simulink model "FYI_Twin_CyberResilient"  (R2025b)
settings: Solver=VariableStepAuto  StartTime=0.0  StopTime=TF  FixedStep=1/120  RelTol=1e-5
PreLoadFcn:
  | [aircraft, state] = astDehavillandBeaver();
  | thrustX = getCoefficient(aircraft,"CX","Propeller",Component="Propeller");
model workspace (MATLAB code in the model file + MAT data in the model file):
  ActuatorCmds = [0.0013469; -0.14185; -0.03733]
  AileronCmd = 0.0013469
  ElevatorCmd = -0.14185
  RudderCmd = -0.03733
  TF = 60
  ThrottleCmd = 0.5
  U0 = 33.0529
  V0 = 0.093272
  W0 = 10.1004
  Xe0 = -2.8165e-12
  Ye0 = 4.3033e-12
  Ze0 = -2202
  aircraft = Aero.FixedWing
  aircraft.ReferenceArea = 23.23
  aircraft.ReferenceSpan = 14.63
  aircraft.ReferenceLength = 1.5875
  aircraft.Coefficients = Aero.FixedWing.Coefficient
  aircraft.Coefficients.Values = {-0.0355, 0, 0.0029, 0, 0, 0, 0, 0, 0, 5.459, -5.162, 0, 0, -0.6748, 0, 0; -0.0022, 0, 0, 0, 0, -0.7678, 0, 0, 0, 0, 0, 0, 0, 0, -0.124, 0.3666; -0.055, 0, -5.578, 0, 0, 0, 0, 0, 0, 0, 3.442, 0, 0, -2.988, 0, 0; 0.000591, 0, 0, 0, 0, -0.0618, 0, 0, 0, 0, 0, 0, 0, 0, -0.5045, 0.1695; 0.0945, 0, -0.6028, 0, 0, 0, 0, 0, 0, -2.14, 0, 0.6921, 0, -15.56, 0, -0.3118; -0.0031, 0, 0, 0, 0, 0.0067, 0, 0, 0, 0, 0, 0, 0.1373, 0.1595, -0.1585, -0.1112}
  aircraft.Coefficients.ReferenceFrame = "Body"
  aircraft.Coefficients.StateVariablesInternal = ["Zero" "U" "Alpha" "AlphaDot" "Q" "Beta" "BetaDot" "P" "R" "Alpha2" "Alpha3" "Beta2" "Beta3" "qcV" "pb2V" "rb2V"]
  aircraft.Surfaces(1) = Aero.FixedWing.Surface
  aircraft.Surfaces(1).Surfaces(1) = Aero.FixedWing.Surface
  aircraft.Surfaces(1).Surfaces(1).Coefficients = Aero.FixedWing.Coefficient
  aircraft.Surfaces(1).Surfaces(1).Coefficients.Values = {0, 0; -0.0296, 0; 0, 0; -0.0992, -0.0827; 0, 0; -0.0039, 0}
  aircraft.Surfaces(1).Surfaces(1).Coefficients.ReferenceFrame = "Body"
  aircraft.Surfaces(1).Surfaces(1).Coefficients.StateVariablesInternal = ["Aileron" "AileronAlpha"]
  aircraft.Surfaces(1).Surfaces(1).MaximumValue = 0.523598775598
  aircraft.Surfaces(1).Surfaces(1).MinimumValue = -0.523598775598
  aircraft.Surfaces(1).Surfaces(1).Symmetry = "Symmetric"
  aircraft.Surfaces(1).Surfaces(1).Properties = Aero.Aircraft.Properties
  aircraft.Surfaces(1).Surfaces(1).Properties.Name = "Aileron"
  aircraft.Surfaces(1).Surfaces(2) = Aero.FixedWing.Surface
  aircraft.Surfaces(1).Surfaces(2).Coefficients = Aero.FixedWing.Coefficient
  aircraft.Surfaces(1).Surfaces(2).Coefficients.Values = {-0.0945, 1.106; 0, 0; -1.377, -1.261; 0, 0; 0.4072, 0; 0, 0}
  aircraft.Surfaces(1).Surfaces(2).Coefficients.ReferenceFrame = "Body"
  aircraft.Surfaces(1).Surfaces(2).Coefficients.StateVariablesInternal = ["Flap" "FlapAlpha"]
  aircraft.Surfaces(1).Surfaces(2).MaximumValue = 0.523598775598
  aircraft.Surfaces(1).Surfaces(2).MinimumValue = -0.523598775598
  aircraft.Surfaces(1).Surfaces(2).Symmetry = "Symmetric"
  aircraft.Surfaces(1).Surfaces(2).Properties = Aero.Aircraft.Properties
  aircraft.Surfaces(1).Surfaces(2).Properties.Name = "Flap"
  aircraft.Surfaces(1).Controllable : enumeration (value not decoded)
  aircraft.Surfaces(1).Symmetry = "Symmetric"
  aircraft.Surfaces(1).Properties = Aero.Aircraft.Properties
  aircraft.Surfaces(1).Properties.Name = "Wing"
  aircraft.Surfaces(2) = Aero.FixedWing.Surface
  aircraft.Surfaces(2).Surfaces = Aero.FixedWing.Surface
  aircraft.Surfaces(2).Surfaces.Coefficients = Aero.FixedWing.Coefficient
  aircraft.Surfaces(2).Surfaces.Coefficients.Values = {0, 0; 0, 0; -0.398, -15.93; 0, 0; -1.921, 0; 0, 0}
  aircraft.Surfaces(2).Surfaces.Coefficients.ReferenceFrame = "Body"
  aircraft.Surfaces(2).Surfaces.Coefficients.StateVariablesInternal = ["Elevator" "ElevatorBeta2"]
  aircraft.Surfaces(2).Surfaces.MaximumValue = 0.523598775598
  aircraft.Surfaces(2).Surfaces.MinimumValue = -0.523598775598
  aircraft.Surfaces(2).Surfaces.Symmetry = "Symmetric"
  aircraft.Surfaces(2).Surfaces.Properties = Aero.Aircraft.Properties
  aircraft.Surfaces(2).Surfaces.Properties.Name = "Elevator"
  aircraft.Surfaces(2).Controllable : enumeration (value not decoded)
  aircraft.Surfaces(2).Symmetry = "Symmetric"
  aircraft.Surfaces(2).Properties = Aero.Aircraft.Properties
  aircraft.Surfaces(2).Properties.Name = "HorizontalStabilizer"
  aircraft.Surfaces(3) = Aero.FixedWing.Surface
  aircraft.Surfaces(3).Surfaces = Aero.FixedWing.Surface
  aircraft.Surfaces(3).Surfaces.Coefficients = Aero.FixedWing.Coefficient
  aircraft.Surfaces(3).Surfaces.Coefficients.Values = {0.0341, 0; 0.1158, 0.5238; 0, 0; 0.0069, 0; 0, 0; -0.0827, 0}
  aircraft.Surfaces(3).Surfaces.Coefficients.ReferenceFrame = "Body"
  aircraft.Surfaces(3).Surfaces.Coefficients.StateVariablesInternal = ["Rudder" "RudderAlpha"]
  aircraft.Surfaces(3).Surfaces.MaximumValue = 1.0471975512
  aircraft.Surfaces(3).Surfaces.MinimumValue = -1.0471975512
  aircraft.Surfaces(3).Surfaces.Symmetry = "Symmetric"
  aircraft.Surfaces(3).Surfaces.Properties = Aero.Aircraft.Properties
  aircraft.Surfaces(3).Surfaces.Properties.Name = "Rudder"
  aircraft.Surfaces(3).Controllable : enumeration (value not decoded)
  aircraft.Surfaces(3).Symmetry = "Symmetric"
  aircraft.Surfaces(3).Properties = Aero.Aircraft.Properties
  aircraft.Surfaces(3).Properties.Name = "VerticalStabilizer"
  aircraft.Thrusts = Aero.FixedWing.Thrust
  aircraft.Thrusts.Coefficients = Aero.FixedWing.Coefficient
  aircraft.Thrusts.Coefficients.Values{1} = Simulink.LookupTable
  aircraft.Thrusts.Coefficients.Values{1}.Table = Simulink.lookuptable.Table
  aircraft.Thrusts.Coefficients.Values{1}.Table.Value = [11.3740665205 82.7365658256 548.333441302 2300 4051.6665587 4517.26343417 4588.62593348]
  aircraft.Thrusts.Coefficients.Values{1}.Table.Dimensions = [1 7]
  aircraft.Thrusts.Coefficients.Values{1}.Table.DataType = 'auto'
  aircraft.Thrusts.Coefficients.Values{1}.Table.FieldName = 'Table'
  aircraft.Thrusts.Coefficients.Values{1}.Breakpoints = Simulink.lookuptable.Breakpoint
  aircraft.Thrusts.Coefficients.Values{1}.Breakpoints.Value = [0 0.166666666667 0.333333333333 0.5 0.666666666667 0.833333333333 1]
  aircraft.Thrusts.Coefficients.Values{1}.Breakpoints.TunableSizeName = 'N1'
  aircraft.Thrusts.Coefficients.Values{1}.Breakpoints.TunableSizeValue = -1
  aircraft.Thrusts.Coefficients.Values{1}.Breakpoints.Dimensions = [1 7]
  aircraft.Thrusts.Coefficients.Values{1}.Breakpoints.DataType = 'auto'
  aircraft.Thrusts.Coefficients.Values{1}.Breakpoints.FieldName = 'Propeller'
  aircraft.Thrusts.Coefficients.Values{1}.AllowMultipleInstancesOfTypeToHaveDifferentTableBreakpointSizes = 0
  aircraft.Thrusts.Coefficients.Values{1}.SupportTunableSize = 0
  aircraft.Thrusts.Coefficients.Values{1}.StructTypeInfo = Simulink.lookuptable.StructTypeInfo
  aircraft.Thrusts.Coefficients.Values{1}.StructTypeInfo.Name = 'Dehavilland_Beaver_Propeller_CX_Propeller'
  aircraft.Thrusts.Coefficients.Values{1}.StructTypeInfo.DataScope = 'Auto'
  aircraft.Thrusts.Coefficients.Values{2} = 0
  aircraft.Thrusts.Coefficients.Values{3} = 0
  aircraft.Thrusts.Coefficients.Values{4} = 0
  aircraft.Thrusts.Coefficients.Values{5} = 0
  aircraft.Thrusts.Coefficients.Values{6} = 0
  aircraft.Thrusts.Coefficients.ReferenceFrame = "Body"
  aircraft.Thrusts.Coefficients.MultiplyStateVariables : enumeration (value not decoded)
  aircraft.Thrusts.Coefficients.NonDimensional : enumeration (value not decoded)
  aircraft.Thrusts.Coefficients.StateVariablesInternal = "Propeller"
  aircraft.Thrusts.MaximumValue = 1
  aircraft.Thrusts.MinimumValue = 0
  aircraft.Thrusts.Symmetry = "Symmetric"
  aircraft.Thrusts.Properties = Aero.Aircraft.Properties
  aircraft.Thrusts.Properties.Name = "Propeller"
  aircraft.Properties = Aero.Aircraft.Properties
  aircraft.Properties.Name = "Dehavilland_Beaver"
  aircraft.Properties.Description = "Dehavilland Beaver demo"
  aircraft.Properties.Type = "General Aviation"
  aircraft.Properties.Version = "1.0"
  aircraft.TemperatureSystem = "Kelvin"
  altitude0 = 2202
  attack_enable = 1
  attack_mode = 3
  blend_rate = 0.05
  inputs0.time = 0
  inputs0.signals(1).dimensions = 1
  inputs0.signals(1).values = -0.104711430294
  inputs0.signals(2).dimensions = 1
  inputs0.signals(2).values = -0.0698725229544
  inputs0.signals(3).dimensions = 1
  inputs0.signals(3).values = -0.000215042330254
  lat0 = 0.843936506509
  lat0_deg = 48.354
  lon0 = 0.205746393542
  lon0_deg = 11.7884
  p0 = 3.0707e-20
  phi0 = 0.0092342
  psi0 = 0
  q0 = 5.1124e-22
  r0 = -8.6217e-20
  required_count = 5
  state = astDehavillandBeaverState
  state.Mass = 2288.231
  state.Inertia = table
  state.Inertia.data = {[5788; 0; -117.6], [0; 6928.9; 0], [117.6; 0; 11578.3]}
  state.Inertia.ndims = 2
  state.Inertia.nrows = 3
  state.Inertia.rownames = {'X'; 'Y'; 'Z'}
  state.Inertia.nvars = 3
  state.Inertia.varnames = {'X', 'Y', 'Z'}
  state.Inertia.props.CustomProps = struct()
  state.Inertia.props.VariableCustomProps = struct()
  state.Inertia.props.versionSavedFrom = 5
  state.Inertia.props.minCompatibleVersion = 1
  state.Inertia.props.incompatibilityMsg = ''
  state.Inertia.props.VersionSavedFrom = 5
  state.Inertia.props.useVariableNamesOriginal = 0
  state.Inertia.props.useVariableNames2048 = 0
  state.Inertia.props.useDimensionNamesOriginal = 0
  state.Inertia.props.useDimensionNames2048 = 0
  state.Inertia.props.Description = ''
  state.Inertia.props.VariableNamesOriginal = {}
  state.Inertia.props.VariableNames2048 = {}
  state.Inertia.props.DimensionNames = {'Row', 'Variables'}
  state.Inertia.props.DimensionNamesOriginal = {}
  state.Inertia.props.DimensionNames2048 = {}
  state.Inertia.props.UserData = []
  state.Inertia.props.VariableDescriptions = {}
  state.Inertia.props.VariableUnits = {}
  state.Inertia.props.VariableContinuity = {}
  state.AltitudeMSL = 2202
  state.XN = -2.8165e-12
  state.XE = 4.3033e-12
  state.U = 33.0529
  state.V = 0.093272
  state.W = 10.1004
  state.Phi = 0.0092342
  state.Theta = 0.29658
  state.P = 3.0707e-20
  state.Q = 5.1124e-22
  state.R = -8.6217e-20
  state.Environment = Aero.Aircraft.Environment
  state.Environment.Density = 0.986207191626
  state.Environment.Temperature = 273.837
  state.Environment.Pressure = 77521.5580145
  state.Environment.SpeedOfSound = 331.734913638
  state.ControlStates(1) = Aero.Aircraft.ControlState
  state.ControlStates(1).MaximumValue = 0.523598775598
  state.ControlStates(1).MinimumValue = -0.523598775598
  state.ControlStates(1).PositionInternal = 0.0091
  state.ControlStates(1).Properties = Aero.Aircraft.Properties
  state.ControlStates(1).Properties.Name = "Aileron"
  state.ControlStates(2) = Aero.Aircraft.ControlState
  state.ControlStates(2).MaximumValue = 0.523598775598
  state.ControlStates(2).MinimumValue = -0.523598775598
  state.ControlStates(2).Properties = Aero.Aircraft.Properties
  state.ControlStates(2).Properties.Name = "Flap"
  state.ControlStates(3) = Aero.Aircraft.ControlState
  state.ControlStates(3).MaximumValue = 0.523598775598
  state.ControlStates(3).MinimumValue = -0.523598775598
  state.ControlStates(3).PositionInternal = -0.0425
  state.ControlStates(3).Properties = Aero.Aircraft.Properties
  state.ControlStates(3).Properties.Name = "Elevator"
  state.ControlStates(4) = Aero.Aircraft.ControlState
  state.ControlStates(4).MaximumValue = 1.0471975512
  state.ControlStates(4).MinimumValue = -1.0471975512
  state.ControlStates(4).PositionInternal = -0.046
  state.ControlStates(4).Properties = Aero.Aircraft.Properties
  state.ControlStates(4).Properties.Name = "Rudder"
  state.ControlStates(5) = Aero.Aircraft.ControlState
  state.ControlStates(5).MaximumValue = 1
  state.ControlStates(5).MinimumValue = 0
  state.ControlStates(5).DeflectionAngle : enumeration (value not decoded)
  state.ControlStates(5).PositionInternal = 0.5
  state.ControlStates(5).Properties = Aero.Aircraft.Properties
  state.ControlStates(5).Properties.Name = "Propeller"
  state.TemperatureSystem = "Kelvin"
  states.time = 0
  states.signals(1).values = 0
  states.signals(1).dimensions = 1
  states.signals(1).label = 'CSTATE'
  states.signals(1).blockName = 'asb6DOFAirframeTemplate/6DOF EOM/6DOF (Euler Angles)/xe,ye,ze'
  states.signals(1).stateName = 'Xe'
  states.signals(1).inReferencedModel = 0
  states.signals(1).sampleTime = [0 0]
  states.signals(2).values = 0
  states.signals(2).dimensions = 1
  states.signals(2).label = 'CSTATE'
  states.signals(2).blockName = 'asb6DOFAirframeTemplate/6DOF EOM/6DOF (Euler Angles)/xe,ye,ze'
  states.signals(2).stateName = 'Ye'
  states.signals(2).inReferencedModel = 0
  states.signals(2).sampleTime = [0 0]
  states.signals(3).values = -2202
  states.signals(3).dimensions = 1
  states.signals(3).label = 'CSTATE'
  states.signals(3).blockName = 'asb6DOFAirframeTemplate/6DOF EOM/6DOF (Euler Angles)/xe,ye,ze'
  states.signals(3).stateName = 'Ze'
  states.signals(3).inReferencedModel = 0
  states.signals(3).sampleTime = [0 0]
  states.signals(4).values = 0.128665353089
  states.signals(4).dimensions = 1
  states.signals(4).label = 'CSTATE'
  states.signals(4).blockName = 'asb6DOFAirframeTemplate/6DOF EOM/6DOF (Euler Angles)/Calculate DCM &
    | Euler Angles/phi
    | theta
    | psi'
  states.signals(4).stateName = 'phi'
  states.signals(4).inReferencedModel = 0
  states.signals(4).sampleTime = [0 0]
  states.signals(5).values = 0.259337659946
  states.signals(5).dimensions = 1
  states.signals(5).label = 'CSTATE'
  states.signals(5).blockName = 'asb6DOFAirframeTemplate/6DOF EOM/6DOF (Euler Angles)/Calculate DCM &
    | Euler Angles/phi
    | theta
    | psi'
  states.signals(5).stateName = 'theta'
  states.signals(5).inReferencedModel = 0
  states.signals(5).sampleTime = [0 0]
  states.signals(6).values = -0.178947917154
  states.signals(6).dimensions = 1
  states.signals(6).label = 'CSTATE'
  states.signals(6).blockName = 'asb6DOFAirframeTemplate/6DOF EOM/6DOF (Euler Angles)/Calculate DCM &
    | Euler Angles/phi
    | theta
    | psi'
  states.signals(6).stateName = 'psi'
  states.signals(6).inReferencedModel = 0
  states.signals(6).sampleTime = [0 0]
  states.signals(7).values = 36.9119692666
  states.signals(7).dimensions = 1
  states.signals(7).label = 'CSTATE'
  states.signals(7).blockName = 'asb6DOFAirframeTemplate/6DOF EOM/6DOF (Euler Angles)/ub,vb,wb'
  states.signals(7).stateName = 'Ubody'
  states.signals(7).inReferencedModel = 0
  states.signals(7).sampleTime = [0 0]
  states.signals(8).values = 8.10720863264
  states.signals(8).dimensions = 1
  states.signals(8).label = 'CSTATE'
  states.signals(8).blockName = 'asb6DOFAirframeTemplate/6DOF EOM/6DOF (Euler Angles)/ub,vb,wb'
  states.signals(8).stateName = 'Vbody'
  states.signals(8).inReferencedModel = 0
  states.signals(8).sampleTime = [0 0]
  states.signals(9).values = 8.82591882596
  states.signals(9).dimensions = 1
  states.signals(9).label = 'CSTATE'
  states.signals(9).blockName = 'asb6DOFAirframeTemplate/6DOF EOM/6DOF (Euler Angles)/ub,vb,wb'
  states.signals(9).stateName = 'Wbody'
  states.signals(9).inReferencedModel = 0
  states.signals(9).sampleTime = [0 0]
  states.signals(10).values = 0
  states.signals(10).dimensions = 1
  states.signals(10).label = 'CSTATE'
  states.signals(10).blockName = 'asb6DOFAirframeTemplate/6DOF EOM/6DOF (Euler Angles)/p,q,r '
  states.signals(10).stateName = 'p'
  states.signals(10).inReferencedModel = 0
  states.signals(10).sampleTime = [0 0]
  states.signals(11).values = 0
  states.signals(11).dimensions = 1
  states.signals(11).label = 'CSTATE'
  states.signals(11).blockName = 'asb6DOFAirframeTemplate/6DOF EOM/6DOF (Euler Angles)/p,q,r '
  states.signals(11).stateName = 'q'
  states.signals(11).inReferencedModel = 0
  states.signals(11).sampleTime = [0 0]
  states.signals(12).values = 0
  states.signals(12).dimensions = 1
  states.signals(12).label = 'CSTATE'
  states.signals(12).blockName = 'asb6DOFAirframeTemplate/6DOF EOM/6DOF (Euler Angles)/p,q,r '
  states.signals(12).stateName = 'r'
  states.signals(12).inReferencedModel = 0
  states.signals(12).sampleTime = [0 0]
  states.signals(13).values = [0 0]
  states.signals(13).dimensions = 2
  states.signals(13).label = 'CSTATE'
  states.signals(13).blockName = 'asb6DOFAirframeTemplate/Environment Model/Dryden Wind Turbulence Model 
    | (Continuous (+q +r))/Filters on velocities/Hwgw(s)/wg_p1'
  states.signals(13).stateName = ''
  states.signals(13).inReferencedModel = 0
  states.signals(13).sampleTime = [0 0]
  states.signals(14).values = [0 0]
  states.signals(14).dimensions = 2
  states.signals(14).label = 'CSTATE'
  states.signals(14).blockName = 'asb6DOFAirframeTemplate/Environment Model/Dryden Wind Turbulence Model 
    | (Continuous (+q +r))/Filters on velocities/Hwgw(s)/wg_p2'
  states.signals(14).stateName = ''
  states.signals(14).inReferencedModel = 0
  states.signals(14).sampleTime = [0 0]
  states.signals(15).values = [0 0]
  states.signals(15).dimensions = 2
  states.signals(15).label = 'CSTATE'
  states.signals(15).blockName = 'asb6DOFAirframeTemplate/Environment Model/Dryden Wind Turbulence Model 
    | (Continuous (+q +r))/Filters on velocities/Hvgw(s)/vg_p1'
  states.signals(15).stateName = ''
  states.signals(15).inReferencedModel = 0
  states.signals(15).sampleTime = [0 0]
  states.signals(16).values = [0 0]
  states.signals(16).dimensions = 2
  states.signals(16).label = 'CSTATE'
  states.signals(16).blockName = 'asb6DOFAirframeTemplate/Environment Model/Dryden Wind Turbulence Model 
    | (Continuous (+q +r))/Filters on velocities/Hvgw(s)/vgw_p2'
  states.signals(16).stateName = ''
  states.signals(16).inReferencedModel = 0
  states.signals(16).sampleTime = [0 0]
  states.signals(17).values = [0 0]
  states.signals(17).dimensions = 2
  states.signals(17).label = 'CSTATE'
  states.signals(17).blockName = 'asb6DOFAirframeTemplate/Environment Model/Dryden Wind Turbulence Model 
    | (Continuous (+q +r))/Filters on velocities/Hugw(s)/ug_p'
  states.signals(17).stateName = ''
  states.signals(17).inReferencedModel = 0
  states.signals(17).sampleTime = [0 0]
  states.signals(18).values = [0 0]
  states.signals(18).dimensions = 2
  states.signals(18).label = 'CSTATE'
  states.signals(18).blockName = 'asb6DOFAirframeTemplate/Environment Model/Dryden Wind Turbulence Model 
    | (Continuous (+q +r))/Filters on angular rates/Hrgw/rgw_p'
  states.signals(18).stateName = ''
  states.signals(18).inReferencedModel = 0
  states.signals(18).sampleTime = [0 0]
  states.signals(19).values = [0 0]
  states.signals(19).dimensions = 2
  states.signals(19).label = 'CSTATE'
  states.signals(19).blockName = 'asb6DOFAirframeTemplate/Environment Model/Dryden Wind Turbulence Model 
    | (Continuous (+q +r))/Filters on angular rates/Hqgw/qgw_p'
  states.signals(19).stateName = ''
  states.signals(19).inReferencedModel = 0
  states.signals(19).sampleTime = [0 0]
  states.signals(20).values = [0 0]
  states.signals(20).dimensions = 2
  states.signals(20).label = 'CSTATE'
  states.signals(20).blockName = 'asb6DOFAirframeTemplate/Environment Model/Dryden Wind Turbulence Model 
    | (Continuous (+q +r))/Filters on angular rates/Hpgw/pgw_p'
  states.signals(20).stateName = ''
  states.signals(20).inReferencedModel = 0
  states.signals(20).sampleTime = [0 0]
  states0.time = 0
  states0.signals(1).values = [0 0 -2202]
  states0.signals(1).dimensions = 3
  states0.signals(1).label = 'CSTATE'
  states0.signals(1).blockName = 'asb6DOFAirframeTemplate/6DOF EOM/6DOF (Euler Angles)/xe,ye,ze'
  states0.signals(1).stateName = ''
  states0.signals(1).inReferencedModel = 0
  states0.signals(1).sampleTime = [0 0]
  states0.signals(2).values = [0.128665353089 0.259337659946 -0.178947917154]
  states0.signals(2).dimensions = 3
  states0.signals(2).label = 'CSTATE'
  states0.signals(2).blockName = 'asb6DOFAirframeTemplate/6DOF EOM/6DOF (Euler Angles)/Calculate DCM &
    | Euler Angles/phi
    | theta
    | psi'
  states0.signals(2).stateName = ''
  states0.signals(2).inReferencedModel = 0
  states0.signals(2).sampleTime = [0 0]
  states0.signals(3).values = [36.9119692666 8.10720863264 8.82591882596]
  states0.signals(3).dimensions = 3
  states0.signals(3).label = 'CSTATE'
  states0.signals(3).blockName = 'asb6DOFAirframeTemplate/6DOF EOM/6DOF (Euler Angles)/ub,vb,wb'
  states0.signals(3).stateName = ''
  states0.signals(3).inReferencedModel = 0
  states0.signals(3).sampleTime = [0 0]
  states0.signals(4).values = [0 0 0]
  states0.signals(4).dimensions = 3
  states0.signals(4).label = 'CSTATE'
  states0.signals(4).blockName = 'asb6DOFAirframeTemplate/6DOF EOM/6DOF (Euler Angles)/p,q,r '
  states0.signals(4).stateName = ''
  states0.signals(4).inReferencedModel = 0
  states0.signals(4).sampleTime = [0 0]
  states0.signals(5).values = [0 0]
  states0.signals(5).dimensions = 2
  states0.signals(5).label = 'CSTATE'
  states0.signals(5).blockName = 'asb6DOFAirframeTemplate/Environment Model/Dryden Wind Turbulence Model 
    | (Continuous (+q +r))/Filters on velocities/Hwgw(s)/wg_p1'
  states0.signals(5).stateName = ''
  states0.signals(5).inReferencedModel = 0
  states0.signals(5).sampleTime = [0 0]
  states0.signals(6).values = [0 0]
  states0.signals(6).dimensions = 2
  states0.signals(6).label = 'CSTATE'
  states0.signals(6).blockName = 'asb6DOFAirframeTemplate/Environment Model/Dryden Wind Turbulence Model 
    | (Continuous (+q +r))/Filters on velocities/Hwgw(s)/wg_p2'
  states0.signals(6).stateName = ''
  states0.signals(6).inReferencedModel = 0
  states0.signals(6).sampleTime = [0 0]
  states0.signals(7).values = [0 0]
  states0.signals(7).dimensions = 2
  states0.signals(7).label = 'CSTATE'
  states0.signals(7).blockName = 'asb6DOFAirframeTemplate/Environment Model/Dryden Wind Turbulence Model 
    | (Continuous (+q +r))/Filters on velocities/Hvgw(s)/vg_p1'
  states0.signals(7).stateName = ''
  states0.signals(7).inReferencedModel = 0
  states0.signals(7).sampleTime = [0 0]
  states0.signals(8).values = [0 0]
  states0.signals(8).dimensions = 2
  states0.signals(8).label = 'CSTATE'
  states0.signals(8).blockName = 'asb6DOFAirframeTemplate/Environment Model/Dryden Wind Turbulence Model 
    | (Continuous (+q +r))/Filters on velocities/Hvgw(s)/vgw_p2'
  states0.signals(8).stateName = ''
  states0.signals(8).inReferencedModel = 0
  states0.signals(8).sampleTime = [0 0]
  states0.signals(9).values = [0 0]
  states0.signals(9).dimensions = 2
  states0.signals(9).label = 'CSTATE'
  states0.signals(9).blockName = 'asb6DOFAirframeTemplate/Environment Model/Dryden Wind Turbulence Model 
    | (Continuous (+q +r))/Filters on velocities/Hugw(s)/ug_p'
  states0.signals(9).stateName = ''
  states0.signals(9).inReferencedModel = 0
  states0.signals(9).sampleTime = [0 0]
  states0.signals(10).values = [0 0]
  states0.signals(10).dimensions = 2
  states0.signals(10).label = 'CSTATE'
  states0.signals(10).blockName = 'asb6DOFAirframeTemplate/Environment Model/Dryden Wind Turbulence Model 
    | (Continuous (+q +r))/Filters on angular rates/Hrgw/rgw_p'
  states0.signals(10).stateName = ''
  states0.signals(10).inReferencedModel = 0
  states0.signals(10).sampleTime = [0 0]
  states0.signals(11).values = [0 0]
  states0.signals(11).dimensions = 2
  states0.signals(11).label = 'CSTATE'
  states0.signals(11).blockName = 'asb6DOFAirframeTemplate/Environment Model/Dryden Wind Turbulence Model 
    | (Continuous (+q +r))/Filters on angular rates/Hqgw/qgw_p'
  states0.signals(11).stateName = ''
  states0.signals(11).inReferencedModel = 0
  states0.signals(11).sampleTime = [0 0]
  states0.signals(12).values = [0 0]
  states0.signals(12).dimensions = 2
  states0.signals(12).label = 'CSTATE'
  states0.signals(12).blockName = 'asb6DOFAirframeTemplate/Environment Model/Dryden Wind Turbulence Model 
    | (Continuous (+q +r))/Filters on angular rates/Hpgw/pgw_p'
  states0.signals(12).stateName = ''
  states0.signals(12).inReferencedModel = 0
  states0.signals(12).sampleTime = [0 0]
  theta0 = 0.29658
  thrustX = Simulink.LookupTable
  thrustX.Table = Simulink.lookuptable.Table
  thrustX.Table.Value = [11.3740665205 82.7365658256 548.333441302 2300 4051.6665587 4517.26343417 4588.62593348]
  thrustX.Table.Dimensions = [1 7]
  thrustX.Table.DataType = 'auto'
  thrustX.Table.FieldName = 'Table'
  thrustX.Breakpoints = Simulink.lookuptable.Breakpoint
  thrustX.Breakpoints.Value = [0 0.166666666667 0.333333333333 0.5 0.666666666667 0.833333333333 1]
  thrustX.Breakpoints.TunableSizeName = 'N1'
  thrustX.Breakpoints.TunableSizeValue = -1
  thrustX.Breakpoints.Dimensions = [1 7]
  thrustX.Breakpoints.DataType = 'auto'
  thrustX.Breakpoints.FieldName = 'Propeller'
  thrustX.AllowMultipleInstancesOfTypeToHaveDifferentTableBreakpointSizes = 0
  thrustX.SupportTunableSize = 0
  thrustX.StructTypeInfo = Simulink.lookuptable.StructTypeInfo
  thrustX.StructTypeInfo.Name = 'Dehavilland_Beaver_Propeller_CX_Propeller'
  thrustX.StructTypeInfo.DataScope = 'Auto'
  u_twin = [0.0013469; -0.14185; -0.03733; 0.5; 0.5]
  x0 = [0.0092342; 0.29658; 0; 3.0707e-20; 5.1124e-22; -8.6217e-20; 33.0529; 0.093272; 10.1004; -2.8165e-12; 4.3033e-12; -2202]
  x0_beaver = [0.0092342; 0.29658; 0; 3.0707e-20; 5.1124e-22; -8.6217e-20; 33.0529; 0.093272; 10.1004; -2.8165e-12; 4.3033e-12; -8202]
  x0_unified = [33.0529; 0.093272; 10.1004; 0.0092342; 0.29658; 0; 3.0707e-20; 5.1124e-22; -8.6217e-20; 0.205746393542; 0.843936506509; 2202]
  other statements: initialize6DOFSkyHogg;
undefined symbols (not defined in the file or in its folder): F, Light, MIL
libraries: aerolibasang x6, aerolibobsolete x2, aerolibadyn x2, aerolibatmos2 x2, aerolibwind2 x2, sharedtransform x2, aerolibfltsims x2
(part 1 of 2)
settings Model: Creator=admin2025  LastModifiedBy=admin2025
settings SolverCC: AlgebraicLoopSolver=TrustRegion  AutoInsertRateTranBlk=on  InsertRTBMode=Never (minimum delay)  MinimalZcImpactIntegration=on  MaxZcPerStep=1.0
settings DataIOCC: ExternalInput=inputs0  InitialState=states  SaveFormat=Array  SaveOutput=off
settings OptimizationCC: BlockReduction=off  EnhancedBackFolding=on  StrengthReduction=on  InitFltsAndDblsToZero=on  DifferentSizesBufferReuse=on
settings DebuggingCC: WriteAfterWriteMsg=DisableAll  AlgebraicLoopMsg=none  FcnCallInpInsideContextMsg=warning  UniqueDataStoreMsg=error  RootOutportRequireBusObject=none  StateNameClashWarn=warning  StrictBusMsg=ErrorOnBusTreatedAsVector  SFUnexpectedBacktrackingDiag=warning  SFNoUnconditionalDefaultTransitionDiag=warning  SFExecutionAtInitializationDiag=none  ArithmeticOperatorsInVariantConditions=warning
settings ModelReferenceCC: EnableRefExpFcnMdlSchedulingChecks=on  PropagateSignalLabelsOutOfModel=off
settings SFSimCC: SimUseLocalCustomCode=off
settings RTWCC: RTWUseLocalCustomCode=off  GPUComputeCapability=3.5  DLArmComputeVersion=19.05
settings CodeAppCC: StateflowObjectComments=on

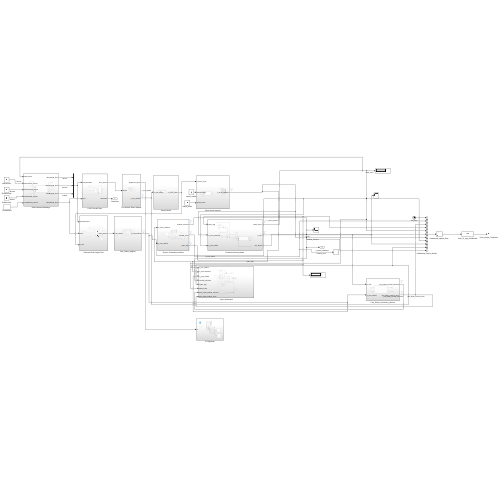
[thumbnail: Simulink's stored preview of the top-level diagram]
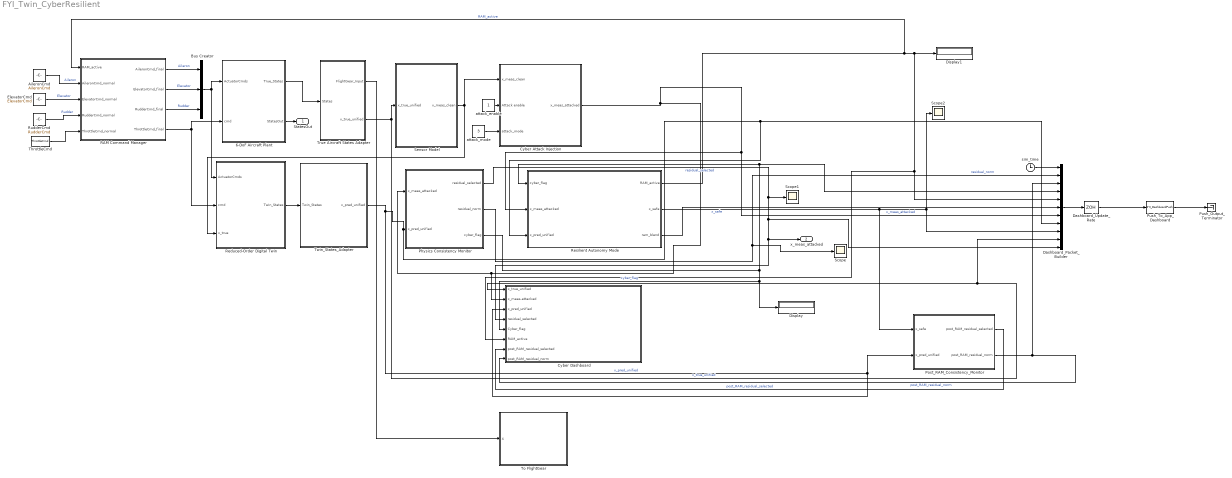
== system FYI_Twin_CyberResilient ==
  6-DoF Aircraft Plant : Subsystem
  AileronCmd : Constant  Value=AileronCmd
  Bus Creator : BusCreator  Inputs=3
  Cyber Attack Injection : Subsystem
  Cyber Dashboard : Subsystem
  Dashboard_Packet_Builder : Concatenate  NumInputs=11
  Dashboard_Update_Rate : ZeroOrderHold  SampleTime=0.1
  Display : Display
  Display1 : Display
  ElevatorCmd : Constant  Value=ElevatorCmd
  Physics Consistency Monitor : Subsystem
  Post_RAM_Consistency_Monitor : Subsystem
  Push_Output_Terminator : Terminator
  Push_To_App_Dashboard : MATLABFcn  MATLABFcn=FYI_DashboardPush
  RAM Command Manager : Subsystem
  Reduced-Order Digital Twin : Subsystem
  Resilient Autonomy Mode : Subsystem
  RudderCmd : Constant  Value=RudderCmd
  Scope : Scope
      settings: ActiveDisplayYMinimum=-76.842271512465658  ActiveDisplayYMaximum=252.07105432729637
  Scope1 : Scope
      settings: ActiveDisplayYMinimum=-7003.9392800862915  ActiveDisplayYMaximum=32762.478212818387  DataLoggingVariableName=ScopeData2
  Scope2 : Scope
      settings: ActiveDisplayYMinimum=-156.7497759524484  ActiveDisplayYMaximum=421.4820575637267  DataLoggingVariableName=ScopeData3
  Sensor Model : Subsystem
  ThrottleCmd : Constant  Value=ThrottleCmd
  To FlightGear : Subsystem
  True Aircraft States Adapter : Subsystem
  Twin_States_Adapter : Subsystem
  attack_enable : Constant
  attack_mode : Constant  Value=3
  sim_time : Clock
  StatesOut : Outport  OutDataTypeStr=double  VectorParamsAs1DForOutWhenUnconnected=off
  x_meas_attacked : Outport  Port=2
  wires:
  6-DoF Aircraft Plant/1(True_States) -> True Aircraft States Adapter/1(States)
  Bus Creator/1 -> 6-DoF Aircraft Plant/1(ActuatorCmds), Reduced-Order Digital Twin/1(ActuatorCmds)
  6-DoF Aircraft Plant/2(StatesOut) -> StatesOut/1
  Sensor Model/1(x_meas_clean) -> Reduced-Order Digital Twin/3(x_true), Cyber Attack Injection/1(x_meas_clean)
  Cyber Attack Injection/1(x_meas_attacked) -> Dashboard_Packet_Builder/7, Resilient Autonomy Mode/2(x_meas_attacked), Physics Consistency Monitor/1(x_meas_attacked), Cyber Dashboard/2(x_meas-attacked)  "x_meas_attacked"
  Physics Consistency Monitor/1(residual_selected) -> Cyber Dashboard/4(residual_selected), x_meas_attacked/1, Dashboard_Packet_Builder/11, Scope1/1  "residual_selected"
  Twin_States_Adapter/1(x_pred_unified) -> Cyber Dashboard/3(x_pred_unified), Post_RAM_Consistency_Monitor/2(x_pred_unified), Dashboard_Packet_Builder/8, Resilient Autonomy Mode/3(x_pred_unified), Physics Consistency Monitor/2(x_pred_unified)  "x_pred_unified"
  True Aircraft States Adapter/2(x_true_unified) -> Sensor Model/1(x_true_unified), Dashboard_Packet_Builder/10, Cyber Dashboard/1(x_true_unified)  "x_true_unified"
  attack_enable/1 -> Cyber Attack Injection/2(Attack enable)
  Physics Consistency Monitor/2(residual_norm) -> Dashboard_Packet_Builder/2, Scope/1  "residual_norm"
  Physics Consistency Monitor/3(cyber_flag) -> Dashboard_Packet_Builder/4, Resilient Autonomy Mode/1(cyber_flag), Display/1, Cyber Dashboard/5(Cyber_flag)  "cyber_flag"
  Resilient Autonomy Mode/2(x_safe) -> Scope2/1, Dashboard_Packet_Builder/9, Post_RAM_Consistency_Monitor/1(x_safe)  "x_safe"
  Resilient Autonomy Mode/1(RAM_active) -> Cyber Dashboard/6(RAM_active), Dashboard_Packet_Builder/5, Display1/1, RAM Command Manager/1(RAM_active)  "RAM_active"
  attack_mode/1 -> Cyber Attack Injection/3(attack_mode)
  AileronCmd/1 -> RAM Command Manager/2(AileronCmd_normal)  "Aileron"
  RAM Command Manager/1(AileronCmd_final) -> Bus Creator/1  "Aileron"
  ElevatorCmd/1 -> RAM Command Manager/3(ElevatorCmd_normal)  "Elevator"
  RAM Command Manager/2(ElevatorCmd_final) -> Bus Creator/2  "Elevator"
  RudderCmd/1 -> RAM Command Manager/4(RudderCmd_normal)  "Rudder"
  ThrottleCmd/1 -> RAM Command Manager/5(ThrottleCmd_normal)
  RAM Command Manager/4(ThrottleCmd_final) -> 6-DoF Aircraft Plant/2(cmd), Reduced-Order Digital Twin/2(cmd)
  Reduced-Order Digital Twin/1(Twin_States) -> Twin_States_Adapter/1(Twin_States)
  RAM Command Manager/3(RudderCmd_final) -> Bus Creator/3  "Rudder"
  Post_RAM_Consistency_Monitor/1(post_RAM_residual_selected) -> Cyber Dashboard/7(post_RAM_residual_selected)  "post_RAM_residual_selected"
  Post_RAM_Consistency_Monitor/2(post_RAM_residual_norm) -> Cyber Dashboard/8(post_RAM_residual_norm), Dashboard_Packet_Builder/3  "post_RAM_residual_norm"
  Resilient Autonomy Mode/3(ram_blend) -> Dashboard_Packet_Builder/6
  sim_time/1 -> Dashboard_Packet_Builder/1
  Dashboard_Packet_Builder/1 -> Dashboard_Update_Rate/1
  Dashboard_Update_Rate/1 -> Push_To_App_Dashboard/1
  Push_To_App_Dashboard/1 -> Push_Output_Terminator/1
  True Aircraft States Adapter/1(FlightGear_Input) -> To FlightGear/1(X)

== system FYI_Twin_CyberResilient/6-DoF Aircraft Plant ==
  ActuatorCmds : Inport
  cmd : Inport  Port=2
  6DOF EOM : Subsystem  VariantControl=eom3DOF
  Aerodynamic Model : Subsystem  VariantControl=aeroCONST
  Environment Model : Subsystem  mask(Environment Model){spec=MIL-F-8785C, model=Continuous Dryden (+q -r), W20=0.005, Wdeg=0, TurbProb=10^-2 - Light, L_high=533.4, Wingspan=4, ts=0.1, Seed=[23341 23342 23343 23344], T_on=on, refAlt=state.GroundHeight}
      mask prompts: spec "aeroblks:aeroblkwind:blockWindTurbulenceModelParamSpecification"; model "aeroblks:aeroblkwind:blockWindTurbulenceModelParamModeltype"; W20 "Wind speed at 6 m defines the low-altitude intensity (m/s):"; Wdeg "Wind direction at 6 m (degrees clockwise from north):"; TurbProb "aeroblks:aeroblkwind:blockWindTurbulenceModelParamProbabilityofexceedanceofhighaltitudeintensity"; L_high "Scale length at medium/high altitudes (m):"; Wingspan "Wingspan (m):"; ts "Band limited noise sample time (sec):"; Seed "aeroblks:aeroblkwind:blockWindTurbulenceModelParamNoiseseedsugvgwgpg"; T_on "aeroblks:aeroblkwind:blockWindTurbulenceModelParamTurbulenceon"; refAlt "Reference height from Earth's surface to Flat Earth frame [m]:"
      mask help: This block contains an athmospheric model, a wind turbulence model, and a gravity model.
      mask Help: helpview(fullfile(docroot,'toolbox','aeroblks','aeroblks.map'), 'environment1');
      mask TypeOptions spec:
      | Dryden Wind Turbulence Model
      | (Continuous (+q +r))/spec
      mask TypeOptions model:
      | Dryden Wind Turbulence Model
      | (Continuous (+q +r))/model
      mask TypeOptions W20:
      | Dryden Wind Turbulence Model
      | (Continuous (+q +r))/W20
      mask TypeOptions Wdeg:
      | Dryden Wind Turbulence Model
      | (Continuous (+q +r))/Wdeg
      mask TypeOptions TurbProb:
      | Dryden Wind Turbulence Model
      | (Continuous (+q +r))/TurbProb
      mask TypeOptions L_high:
      | Dryden Wind Turbulence Model
      | (Continuous (+q +r))/L_high
      mask TypeOptions Wingspan:
      | Dryden Wind Turbulence Model
      | (Continuous (+q +r))/Wingspan
      mask TypeOptions ts:
      | Dryden Wind Turbulence Model
      | (Continuous (+q +r))/ts
      mask TypeOptions Seed:
      | Dryden Wind Turbulence Model
      | (Continuous (+q +r))/Seed
      mask TypeOptions T_on:
      | Dryden Wind Turbulence Model
      | (Continuous (+q +r))/T_on
      mask DialogControl Container4 Prompt: Atmospheric Model
      mask DialogControl Container17 Prompt: 1976 COESA-extended U.S. Standard Atmospheric Model
      mask DialogControl Control6 Prompt: There are no modifiable parameters for COESA.
      mask DialogControl Container6 Prompt: Wind Model
      mask DialogControl Container16 Prompt: Dryden Wind Turbulence Model
      mask DialogControl spec Prompt: Specification:
      mask DialogControl model Prompt: Model type:
      mask DialogControl TurbProb Prompt: Probability of exceedance of high-altitude intensity:
      mask DialogControl Seed Prompt: Noise seeds [ug vg wg pg]:
      mask DialogControl T_on Prompt: Turbulence on
      mask DialogControl Container8 Prompt: Gravity Model
      mask DialogControl Container18 Prompt: World Geodetic System (WGS 84) Gravity Taylor Series Model
      mask Display:
      | image('aeroenvironment.bmp',[.15,.15,.55,.75])
      | port_label('output',1,'Env')
  Propulsion : Subsystem
      settings: RTWSystemCode=Inline
  Sum1 : Sum  Inputs=|++  InputSameDT=on  SaturateOnIntegerOverflow=on  OutDataTypeStr=Inherit: Same as first input
  Sum2 : Sum  Inputs=|++  InputSameDT=on  SaturateOnIntegerOverflow=on  OutDataTypeStr=Inherit: Same as first input
  True_States : Outport
  StatesOut : Outport  Port=2
  wires:
  Aerodynamic Model/1(F) -> Sum2/1
  Aerodynamic Model/2(M) -> Sum1/1
  Environment Model/1(Env) -> Aerodynamic Model/1(Env), 6DOF EOM/1(Env)
  cmd/1 -> Propulsion/1(cmd)
  Propulsion/1(F) -> Sum2/2
  ActuatorCmds/1 -> Aerodynamic Model/2(ActuatorCmds)
  Sum1/1 -> 6DOF EOM/3(Moments)
  Propulsion/2(M) -> Sum1/2
  Sum2/1 -> 6DOF EOM/2(Forces)
  6DOF EOM/1(States) -> Aerodynamic Model/3(States), StatesOut/1, True_States/1, Environment Model/1(States)

== system FYI_Twin_CyberResilient/Cyber Attack Injection ==
  x_meas_clean : Inport
  Attack enable : Inport  Port=2
  attack_mode : Inport  Port=3
  Add : Sum
  Add1 : Sum
  Clock : Clock
  Constant : Constant  Value=0
  Constant1 : Constant  Value=0
  Demux : Demux  Outputs=12
  MATLAB Function : MATLAB Function  TreatAsAtomicUnit=on
  Mux : Mux  Inputs=12
  x_meas_attacked : Outport
  wires:
  Demux/5 -> Mux/5
  Demux/3 -> Mux/3
  Demux/4 -> Mux/4
  Demux/2 -> Mux/2
  Demux/6 -> Mux/6
  Demux/7 -> Mux/7
  Demux/8 -> Mux/8
  Demux/9 -> Mux/9
  Demux/10 -> Mux/10
  Demux/11 -> Mux/11
  Demux/12 -> Add/1
  Add/1 -> Mux/12
  Constant1/1 -> Add/2
  Add1/1 -> Mux/1
  Demux/1 -> Add1/2
  Constant/1 -> Add1/1
  x_meas_clean/1 -> MATLAB Function/1(x_meas_clean)
  MATLAB Function/1(x_meas_attacked) -> x_meas_attacked/1
  Attack enable/1 -> MATLAB Function/2(attack_enable)
  Clock/1 -> MATLAB Function/4(t)
  attack_mode/1 -> MATLAB Function/3(attack_mode)

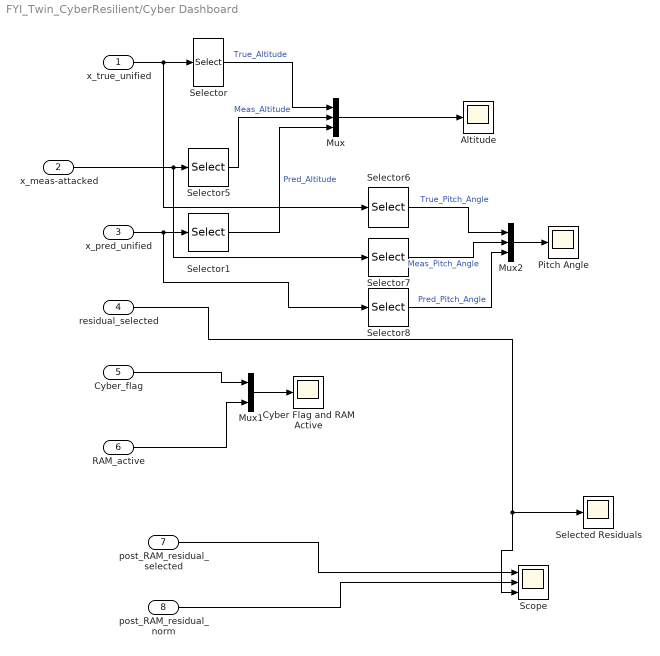
== system FYI_Twin_CyberResilient/Cyber Dashboard ==
  x_true_unified : Inport
  x_meas-attacked : Inport  Port=2
  x_pred_unified : Inport  Port=3
  residual_selected : Inport  Port=4
  Cyber_flag : Inport  Port=5
  RAM_active : Inport  Port=6
  post_RAM_residual_selected : Inport  Port=7
  post_RAM_residual_norm : Inport  Port=8
  Altitude : Scope
      settings: ActiveDisplayYMinimum=43.932530924028782  ActiveDisplayYMaximum=306.83003984343588  YLabel=Altitude (m)  DataLoggingVariableName=ScopeData4
  Cyber Flag and RAM Active : Scope
      settings: ActiveDisplayYMinimum=-0.36825982849504812  ActiveDisplayYMaximum=0.93174017150495159  DataLoggingVariableName=ScopeData6
  Mux : Mux  Inputs=3
  Mux1 : Mux  Inputs=2
  Mux2 : Mux  Inputs=3
  Pitch Angle : Scope
      settings: ActiveDisplayYMinimum=-150.79859392506594  ActiveDisplayYMaximum=371.968487219726  DataLoggingVariableName=ScopeData7
  Scope : Scope  NumInputPorts=3
      settings: ActiveDisplayYMinimum=-3.03100486656035  ActiveDisplayYMaximum=7.0158479530724636  DataLoggingVariableName=ScopeData8
  Selected Residuals : Scope
      settings: ActiveDisplayYMinimum=-1159.9122691629195  ActiveDisplayYMaximum=2451.107618108816  DataLoggingVariableName=ScopeData5
  Selector : Selector  InputPortWidth=12  IndexOptions=Index vector (dialog)  Indices=12  OutputSizes=1
  Selector1 : Selector  InputPortWidth=12  IndexOptions=Index vector (dialog)  Indices=12  OutputSizes=1
  Selector5 : Selector  InputPortWidth=12  IndexOptions=Index vector (dialog)  Indices=12  OutputSizes=1
  Selector6 : Selector  InputPortWidth=12  IndexOptions=Index vector (dialog)  Indices=5  OutputSizes=1
  Selector7 : Selector  InputPortWidth=12  IndexOptions=Index vector (dialog)  Indices=5  OutputSizes=1
  Selector8 : Selector  InputPortWidth=12  IndexOptions=Index vector (dialog)  Indices=5  OutputSizes=1
  wires:
  x_true_unified/1 -> Selector6/1, Selector/1
  x_pred_unified/1 -> Selector8/1, Selector1/1
  x_meas-attacked/1 -> Selector7/1, Selector5/1
  Selector/1 -> Mux/1  "True_Altitude"
  Selector5/1 -> Mux/2  "Meas_Altitude"
  Selector1/1 -> Mux/3  "Pred_Altitude"
  Mux/1 -> Altitude/1
  Mux1/1 -> Cyber Flag and RAM Active/1
  Cyber_flag/1 -> Mux1/1
  RAM_active/1 -> Mux1/2
  residual_selected/1 -> Scope/3, Selected Residuals/1
  Selector6/1 -> Mux2/1  "True_Pitch_Angle"
  Selector7/1 -> Mux2/2  "Meas_Pitch_Angle"
  Selector8/1 -> Mux2/3  "Pred_Pitch_Angle"
  Mux2/1 -> Pitch Angle/1
  post_RAM_residual_selected/1 -> Scope/1
  post_RAM_residual_norm/1 -> Scope/2

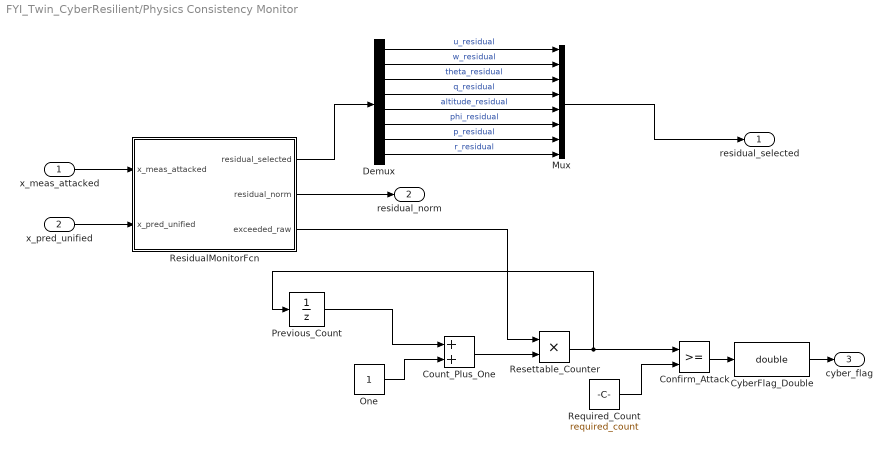
== system FYI_Twin_CyberResilient/Physics Consistency Monitor ==
  x_meas_attacked : Inport
  x_pred_unified : Inport  Port=2
  Confirm_Attack : RelationalOperator  OutDataTypeStr=boolean  RndMeth=Simplest  InputSameDT=off
  Count_Plus_One : Sum
  CyberFlag_Double : DataTypeConversion  OutDataTypeStr=double  SaturateOnIntegerOverflow=off  RndMeth=Floor
  Demux : Demux  Outputs=8
  Mux : Mux  Inputs=8
  One : Constant
  Previous_Count : UnitDelay  SampleTime=0.1  HasFrameUpgradeWarning=on
  Required_Count : Constant  Value=required_count
  Resettable_Counter : Product
  ResidualMonitorFcn : MATLAB Function  TreatAsAtomicUnit=on
  residual_selected : Outport
  residual_norm : Outport  Port=2
  cyber_flag : Outport  Port=3
  wires:
  x_meas_attacked/1 -> ResidualMonitorFcn/1(x_meas_attacked)
  x_pred_unified/1 -> ResidualMonitorFcn/2(x_pred_unified)
  ResidualMonitorFcn/2(residual_norm) -> residual_norm/1
  ResidualMonitorFcn/1(residual_selected) -> Demux/1
  Demux/1 -> Mux/1  "u_residual"
  Demux/2 -> Mux/2  "w_residual"
  Demux/3 -> Mux/3  "theta_residual"
  Demux/4 -> Mux/4  "q_residual"
  Demux/5 -> Mux/5  "altitude_residual"
  Demux/6 -> Mux/6  "phi_residual"
  Demux/7 -> Mux/7  "p_residual"
  Demux/8 -> Mux/8  "r_residual"
  Mux/1 -> residual_selected/1
  One/1 -> Count_Plus_One/2
  Previous_Count/1 -> Count_Plus_One/1
  Count_Plus_One/1 -> Resettable_Counter/2
  ResidualMonitorFcn/3(exceeded_raw) -> Resettable_Counter/1
  Resettable_Counter/1 -> Previous_Count/1, Confirm_Attack/1
  Required_Count/1 -> Confirm_Attack/2
  Confirm_Attack/1 -> CyberFlag_Double/1
  CyberFlag_Double/1 -> cyber_flag/1

== system FYI_Twin_CyberResilient/Post_RAM_Consistency_Monitor ==
  x_safe : Inport
  x_pred_unified : Inport  Port=2
  MATLAB Function : MATLAB Function  TreatAsAtomicUnit=on
  post_RAM_residual_selected : Outport
  post_RAM_residual_norm : Outport  Port=2
  wires:
  x_safe/1 -> MATLAB Function/1(x_safe)
  x_pred_unified/1 -> MATLAB Function/2(x_pred_unified)
  MATLAB Function/1(post_RAM_residual_selected) -> post_RAM_residual_selected/1
  MATLAB Function/2(post_RAM_residual_norm) -> post_RAM_residual_norm/1

== system FYI_Twin_CyberResilient/RAM Command Manager ==
  RAM_active : Inport
  AileronCmd_normal : Inport  Port=2
  ElevatorCmd_normal : Inport  Port=3
  RudderCmd_normal : Inport  Port=4
  ThrottleCmd_normal : Inport  Port=5
  MATLAB Function : MATLAB Function  TreatAsAtomicUnit=on
  AileronCmd_final : Outport
  ElevatorCmd_final : Outport  Port=2
  RudderCmd_final : Outport  Port=3
  ThrottleCmd_final : Outport  Port=4
  wires:
  RAM_active/1 -> MATLAB Function/1(RAM_active)
  AileronCmd_normal/1 -> MATLAB Function/2(aileron_in)
  ElevatorCmd_normal/1 -> MATLAB Function/3(elevator_in)
  RudderCmd_normal/1 -> MATLAB Function/4(rudder_in)
  ThrottleCmd_normal/1 -> MATLAB Function/5(throttle_in)
  MATLAB Function/1(aileron_out) -> AileronCmd_final/1
  MATLAB Function/2(elevator_out) -> ElevatorCmd_final/1
  MATLAB Function/3(rudder_out) -> RudderCmd_final/1
  MATLAB Function/4(throttle_out) -> ThrottleCmd_final/1

== system FYI_Twin_CyberResilient/Reduced-Order Digital Twin ==
  ActuatorCmds : Inport
  cmd : Inport  Port=2
  x_true : Inport  Port=3
  6DOF EOM1 : Subsystem  VariantControl=eom3DOF
  Aerodynamic Model : Subsystem  VariantControl=aeroCONST
  Display : Display
  Display1 : Display
  Environment Model : Subsystem  mask(Environment Model){spec=MIL-F-8785C, model=Continuous Dryden (+q -r), W20=5, Wdeg=0, TurbProb=10^-2 - Light, L_high=533.4, Wingspan=4, ts=0.1, Seed=[23341 23342 23343 23344], T_on=off, refAlt=state.GroundHeight}
      mask prompts: spec "aeroblks:aeroblkwind:blockWindTurbulenceModelParamSpecification"; model "aeroblks:aeroblkwind:blockWindTurbulenceModelParamModeltype"; W20 "Wind speed at 6 m defines the low-altitude intensity (m/s):"; Wdeg "Wind direction at 6 m (degrees clockwise from north):"; TurbProb "aeroblks:aeroblkwind:blockWindTurbulenceModelParamProbabilityofexceedanceofhighaltitudeintensity"; L_high "Scale length at medium/high altitudes (m):"; Wingspan "Wingspan (m):"; ts "Band limited noise sample time (sec):"; Seed "aeroblks:aeroblkwind:blockWindTurbulenceModelParamNoiseseedsugvgwgpg"; T_on "aeroblks:aeroblkwind:blockWindTurbulenceModelParamTurbulenceon"; refAlt "Reference height from Earth's surface to Flat Earth frame [m]:"
      mask help: This block contains an athmospheric model, a wind turbulence model, and a gravity model.
      mask Help: helpview(fullfile(docroot,'toolbox','aeroblks','aeroblks.map'), 'environment1');
      mask TypeOptions spec:
      | Dryden Wind Turbulence Model
      | (Continuous (+q +r))/spec
      mask TypeOptions model:
      | Dryden Wind Turbulence Model
      | (Continuous (+q +r))/model
      mask TypeOptions W20:
      | Dryden Wind Turbulence Model
      | (Continuous (+q +r))/W20
      mask TypeOptions Wdeg:
      | Dryden Wind Turbulence Model
      | (Continuous (+q +r))/Wdeg
      mask TypeOptions TurbProb:
      | Dryden Wind Turbulence Model
      | (Continuous (+q +r))/TurbProb
      mask TypeOptions L_high:
      | Dryden Wind Turbulence Model
      | (Continuous (+q +r))/L_high
      mask TypeOptions Wingspan:
      | Dryden Wind Turbulence Model
      | (Continuous (+q +r))/Wingspan
      mask TypeOptions ts:
      | Dryden Wind Turbulence Model
      | (Continuous (+q +r))/ts
      mask TypeOptions Seed:
      | Dryden Wind Turbulence Model
      | (Continuous (+q +r))/Seed
      mask TypeOptions T_on:
      | Dryden Wind Turbulence Model
      | (Continuous (+q +r))/T_on
      mask DialogControl Container4 Prompt: Atmospheric Model
      mask DialogControl Container17 Prompt: 1976 COESA-extended U.S. Standard Atmospheric Model
      mask DialogControl Control6 Prompt: There are no modifiable parameters for COESA.
      mask DialogControl Container6 Prompt: Wind Model
      mask DialogControl Container16 Prompt: Dryden Wind Turbulence Model
      mask DialogControl spec Prompt: Specification:
      mask DialogControl model Prompt: Model type:
      mask DialogControl TurbProb Prompt: Probability of exceedance of high-altitude intensity:
      mask DialogControl Seed Prompt: Noise seeds [ug vg wg pg]:
      mask DialogControl T_on Prompt: Turbulence on
      mask DialogControl Container8 Prompt: Gravity Model
      mask DialogControl Container18 Prompt: World Geodetic System (WGS 84) Gravity Taylor Series Model
      mask Display:
      | image('aeroenvironment.bmp',[.15,.15,.55,.75])
      | port_label('output',1,'Env')
  Propulsion : Subsystem
      settings: RTWSystemCode=Inline
  Reduced_Twin_Propulsion : MATLAB Function  TreatAsAtomicUnit=on
  Sum1 : Sum  Inputs=|++  InputSameDT=on  SaturateOnIntegerOverflow=on  OutDataTypeStr=Inherit: Same as first input
  Sum2 : Sum  Inputs=|++  InputSameDT=on  SaturateOnIntegerOverflow=on  OutDataTypeStr=Inherit: Same as first input
  Twin_States : Outport
  wires:
  x_true/1 -> ?
  Reduced_Twin_Propulsion/1(F) -> Display/1, Sum2/2
  cmd/1 -> Reduced_Twin_Propulsion/1(cmd)
  ActuatorCmds/1 -> Aerodynamic Model/2(ActuatorCmds)
  Reduced_Twin_Propulsion/2(M) -> Sum1/2, Display1/1
  Aerodynamic Model/1(F) -> Sum2/1
  Aerodynamic Model/2(M) -> Sum1/1
  6DOF EOM1/1(States) -> Twin_States/1, Aerodynamic Model/3(States), Environment Model/1(States)
  Environment Model/1(Env) -> 6DOF EOM1/1(Env), Aerodynamic Model/1(Env)
  Sum2/1 -> 6DOF EOM1/2(Forces)
  Sum1/1 -> 6DOF EOM1/3(Moments)

== system FYI_Twin_CyberResilient/Resilient Autonomy Mode ==
  cyber_flag : Inport
  x_meas_attacked : Inport  Port=2
  x_pred_unified : Inport  Port=3
  Blend_Plus_Rate : Sum
  Blend_Rate : Constant  Value=blend_rate
  Limit_Blend_0_to_1 : Saturate  UpperLimit=1  LowerLimit=0
  Previous_Blend : UnitDelay  SampleTime=0.1  HasFrameUpgradeWarning=on
  RAMLogic : MATLAB Function  TreatAsAtomicUnit=on
  Reset_Blend_When_No_RAM : Product
  RAM_active : Outport
  x_safe : Outport  Port=2
  ram_blend : Outport  Port=3
  wires:
  cyber_flag/1 -> Reset_Blend_When_No_RAM/2, RAMLogic/1(cyber_flag)
  x_meas_attacked/1 -> RAMLogic/3(x_meas_attacked)
  x_pred_unified/1 -> RAMLogic/4(x_pred_unified)
  RAMLogic/1(RAM_active) -> RAM_active/1
  RAMLogic/2(x_safe) -> x_safe/1
  Previous_Blend/1 -> Blend_Plus_Rate/1
  Blend_Rate/1 -> Blend_Plus_Rate/2
  Blend_Plus_Rate/1 -> Limit_Blend_0_to_1/1
  Limit_Blend_0_to_1/1 -> Reset_Blend_When_No_RAM/1
  Reset_Blend_When_No_RAM/1 -> Previous_Blend/1, ram_blend/1, RAMLogic/2(ram_blend)  "ram_blend"

== system FYI_Twin_CyberResilient/Sensor Model ==
  x_true_unified : Inport
  Clock : Clock
  SensorModelFcn : MATLAB Function  TreatAsAtomicUnit=on
  x_meas_clean : Outport
  wires:
  x_true_unified/1 -> SensorModelFcn/1(x_true)
  SensorModelFcn/1(x_meas) -> x_meas_clean/1
  Clock/1 -> SensorModelFcn/2(t)

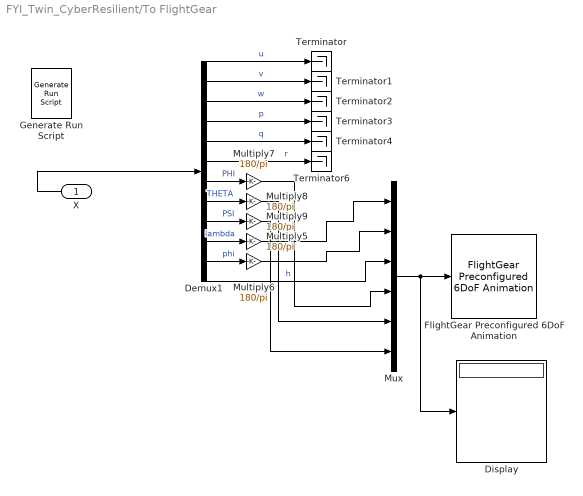
== system FYI_Twin_CyberResilient/To FlightGear ==
  X : Inport
  Demux1 : Demux  Outputs=12
  Display : Display
  FlightGear Preconfigured 6DoF Animation : aerolibfltsims/FlightGear Preconfigured 6DoF Animation  xFlightGearVersion=v2019.1  DestinationIpAddress=127.0.0.1  DestinationPort=5502  SampleTime=1/30  packetVersion=24
  Generate Run Script : aerolibfltsims/Generate Run Script  Architecture=Linux  dataFlow=Send  GeometryModelName=737-300  AirportId=KSFO  RunwayId=10L  InitialAltitude=3000*3.28084  InitialHeading=113  OffsetDistance=4.72  OffsetAzimuth=0  InstallScenery=on  DisableShaders=on  OriginAddress=127.0.0.1  DestinationPort=5502  OriginPort=5505  LocalAddress=127.0.0.1  OutputFileName=runfgt.bat  FlightGearBaseDirectory=C:\Program Files\FlightGear 2024.1
  Multiply{5..9} (5 alike) : Gain  Gain=180/pi
  Mux : Mux  Inputs=6
  Terminator{,1..4,6} (6 alike) : Terminator
  wires:
  Demux1/4 -> Terminator3/1  "p"
  Demux1/10 -> Multiply5/1  "lambda"
  Demux1/7 -> Multiply7/1  "PHI"
  Multiply7/1 -> Mux/4
  Demux1/1 -> Terminator/1  "u"
  Demux1/11 -> Multiply6/1  "phi"
  Demux1/12 -> Mux/3  "h"
  Demux1/9 -> Multiply9/1  "PSI"
  Demux1/8 -> Multiply8/1  "THETA"
  Multiply5/1 -> Mux/1
  Mux/1 -> Display/1, FlightGear Preconfigured 6DoF Animation/1
  Multiply9/1 -> Mux/6
  Demux1/6 -> Terminator6/1  "r"
  Multiply8/1 -> Mux/5
  Demux1/3 -> Terminator2/1  "w"
  Demux1/2 -> Terminator1/1  "v"
  Multiply6/1 -> Mux/2
  Demux1/5 -> Terminator4/1  "q"
  X/1 -> Demux1/1

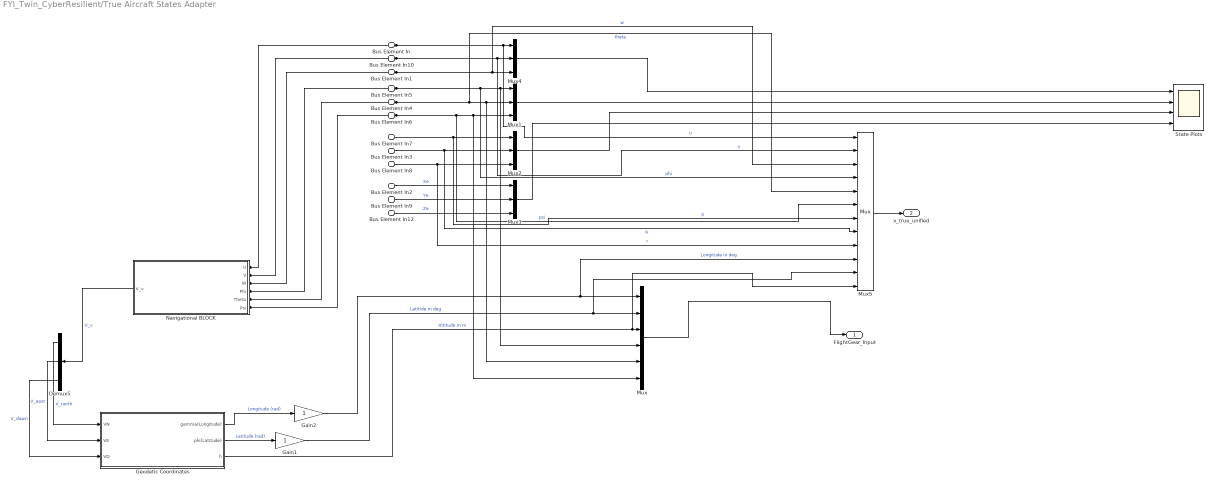
== system FYI_Twin_CyberResilient/True Aircraft States Adapter ==
  Bus Element In : Inport  PortName=States  Element=u
  Bus Element In1 : Inport  PortName=States  Element=w
  Bus Element In3 : Inport  PortName=States  Element=q
  Bus Element In4 : Inport  PortName=States  Element=theta
  Bus Element In12 : Inport  PortName=States  Element=Ze
  Bus Element In2 : Inport  PortName=States  Element=Xe
  Bus Element In10 : Inport  PortName=States  Element=v
  Bus Element In5 : Inport  PortName=States  Element=phi
  Bus Element In6 : Inport  PortName=States  Element=psi
  Bus Element In7 : Inport  PortName=States  Element=p
  Bus Element In8 : Inport  PortName=States  Element=r
  Bus Element In9 : Inport  PortName=States  Element=Ye
  Demux5 : Demux  Outputs=3
  Gain1 : Gain
  Gain2 : Gain
  Geodetic Coordinates : Subsystem
  Mux : Mux  Inputs=6
  Mux{1..4} (4 alike) : Mux  Inputs=3
  Mux5 : Mux  Inputs=12
      settings: DisplayOption=signals
  Navigational BLOCK : Subsystem
  State Plots : Scope  NumInputPorts=4
      settings: ActiveDisplayString=4  Title=Inertial Position vs Time  ActiveDisplayYMinimum=-35273.126798598096  ActiveDisplayYMaximum=9851.523878667198  YLabel=Xe Ye Ze [m]  DataLoggingVariableName=ScopeData9
  FlightGear_Input : Outport
  x_true_unified : Outport  Port=2
  wires:
  Bus Element In2/1 -> Mux3/1  "Xe"
  Bus Element In9/1 -> Mux3/2  "Ye"
  Bus Element In12/1 -> Mux3/3  "Ze"
  Bus Element In8/1 -> Mux5/9, Mux2/3  "r"
  Bus Element In7/1 -> Mux5/7, Mux2/1  "p"
  Bus Element In6/1 -> Mux5/6, Mux1/3, Mux/6, Navigational BLOCK/6(Psi)  "psi"
  Bus Element In5/1 -> Mux5/4, Mux/4, Mux1/1, Navigational BLOCK/4(Phi)  "phi"
  Bus Element In4/1 -> Mux5/5, Mux1/2, Mux/5, Navigational BLOCK/5(Theta)  "theta"
  Bus Element In3/1 -> Mux5/8, Mux2/2  "q"
  Mux/1 -> FlightGear_Input/1
  Geodetic Coordinates/2(phi(Latitude)) -> Gain1/1  "Latitude (rad)"
  Bus Element In1/1 -> Mux5/3, Mux4/3, Navigational BLOCK/3(W)  "w"
  Navigational BLOCK/1(V_v) -> Demux5/1  "V_v"
  Demux5/2 -> Geodetic Coordinates/2(VE)  "V_east"
  Bus Element In10/1 -> Mux5/2, Mux4/2, Navigational BLOCK/2(V)  "v"
  Geodetic Coordinates/3(h) -> Mux5/12, Mux/3  "Altitude in m"
  Bus Element In/1 -> Mux5/1, Mux4/1, Navigational BLOCK/1(U)  "u"
  Demux5/1 -> Geodetic Coordinates/1(VN)  "V_north"
  Demux5/3 -> Geodetic Coordinates/3(VD)  "V_down"
  Geodetic Coordinates/1(gamma(Longitude)) -> Gain2/1  "Longitude (rad)"
  Gain2/1 -> Mux5/10, Mux/1  "Longitude in deg"
  Gain1/1 -> Mux/2, Mux5/11  "Latitide in deg"
  Mux5/1 -> x_true_unified/1
  Mux4/1 -> State Plots/1
  Mux1/1 -> State Plots/2
  Mux2/1 -> State Plots/3
  Mux3/1 -> State Plots/4

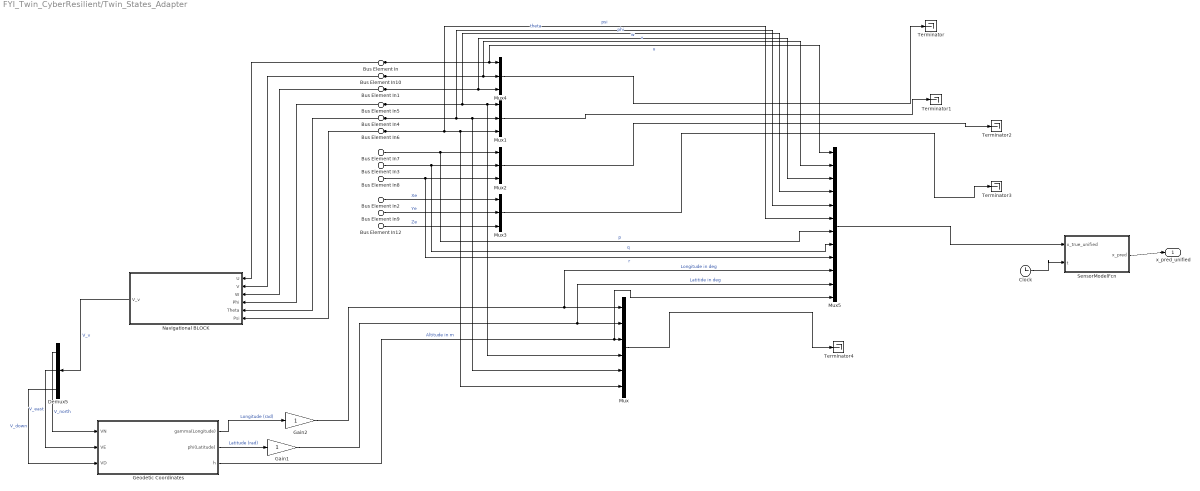
== system FYI_Twin_CyberResilient/Twin_States_Adapter ==
  Bus Element In : Inport  PortName=Twin_States  Element=u
  Bus Element In1 : Inport  PortName=Twin_States  Element=w
  Bus Element In3 : Inport  PortName=Twin_States  Element=q
  Bus Element In4 : Inport  PortName=Twin_States  Element=theta
  Bus Element In12 : Inport  PortName=Twin_States  Element=Ze
  Bus Element In2 : Inport  PortName=Twin_States  Element=Xe
  Bus Element In10 : Inport  PortName=Twin_States  Element=v
  Bus Element In5 : Inport  PortName=Twin_States  Element=phi
  Bus Element In6 : Inport  PortName=Twin_States  Element=psi
  Bus Element In7 : Inport  PortName=Twin_States  Element=p
  Bus Element In8 : Inport  PortName=Twin_States  Element=r
  Bus Element In9 : Inport  PortName=Twin_States  Element=Ye
  Clock : Clock
  Demux5 : Demux  Outputs=3
  Gain1 : Gain
  Gain2 : Gain
  Geodetic Coordinates : Subsystem
  Mux : Mux  Inputs=6
  Mux{1..4} (4 alike) : Mux  Inputs=3
  Mux5 : Mux  Inputs=12
  Navigational BLOCK : Subsystem
  SensorModelFcn : MATLAB Function  TreatAsAtomicUnit=on
  Terminator{,1..4} (5 alike) : Terminator
  x_pred_unified : Outport
  wires:
  Mux3/1 -> Terminator3/1
  Bus Element In2/1 -> Mux3/1  "Xe"
  Bus Element In9/1 -> Mux3/2  "Ye"
  Bus Element In12/1 -> Mux3/3  "Ze"
  Mux2/1 -> Terminator2/1
  Mux1/1 -> Terminator1/1
  Mux4/1 -> Terminator/1
  Bus Element In8/1 -> Mux5/9, Mux2/3  "r"
  Bus Element In7/1 -> Mux5/7, Mux2/1  "p"
  Bus Element In6/1 -> Mux5/6, Mux1/3, Mux/6, Navigational BLOCK/6(Psi)  "psi"
  Bus Element In5/1 -> Mux5/4, Mux/4, Mux1/1, Navigational BLOCK/4(Phi)  "phi"
  Bus Element In4/1 -> Mux5/5, Mux1/2, Mux/5, Navigational BLOCK/5(Theta)  "theta"
  Bus Element In3/1 -> Mux5/8, Mux2/2  "q"
  Mux/1 -> Terminator4/1
  Geodetic Coordinates/2(phi(Latitude)) -> Gain1/1  "Latitude (rad)"
  Bus Element In1/1 -> Mux5/3, Mux4/3, Navigational BLOCK/3(W)  "w"
  Navigational BLOCK/1(V_v) -> Demux5/1  "V_v"
  Demux5/2 -> Geodetic Coordinates/2(VE)  "V_east"
  Bus Element In10/1 -> Mux5/2, Mux4/2, Navigational BLOCK/2(V)  "v"
  Geodetic Coordinates/3(h) -> Mux5/12, Mux/3  "Altitude in m"
  Bus Element In/1 -> Mux5/1, Mux4/1, Navigational BLOCK/1(U)  "u"
  Demux5/1 -> Geodetic Coordinates/1(VN)  "V_north"
  Demux5/3 -> Geodetic Coordinates/3(VD)  "V_down"
  Geodetic Coordinates/1(gamma(Longitude)) -> Gain2/1  "Longitude (rad)"
  Gain2/1 -> Mux5/10, Mux/1  "Longitude in deg"
  Gain1/1 -> Mux/2, Mux5/11  "Latitide in deg"
  Clock/1 -> SensorModelFcn/2(t)
  SensorModelFcn/1(x_pred) -> x_pred_unified/1
  Mux5/1 -> SensorModelFcn/1(x_true_unified)

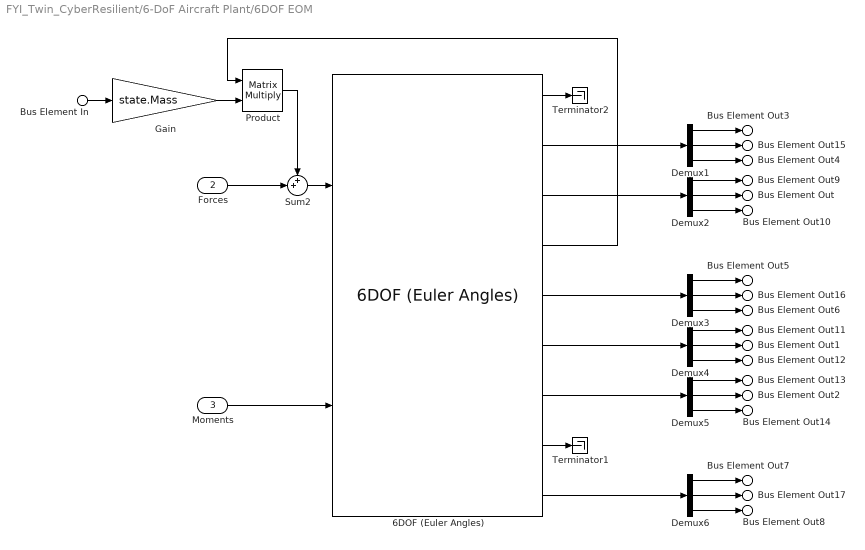
== system FYI_Twin_CyberResilient/6-DoF Aircraft Plant/6DOF EOM ==
  Bus Element In : Inport  PortName=Env  Element=g
  Forces : Inport  Port=2
  Moments : Inport  Port=3
  6DOF (Euler Angles) : aerolibobsolete/6DOF (Euler Angles)  units=Metric (MKS)  mtype=Fixed  rep=Euler Angles  xme_0=[Xe0, Ye0, Ze0]  Vm_0=[U0, V0, W0]  eul_0=[phi0, theta0, psi0]  pm_0=[p0, q0, r0]  mass_0=state.Mass  mass_e=0.5  mass_f=2.0  inertia=state.Inertia.Variables  inertia_e=eye(3)  inertia_f=2*eye(3)  k_quat=1.0  vre_flag=on  abi_flag=on  aMode=0  xme_statename={'Xe', 'Ye', 'Ze'}  Vm_statename={'U', 'V', 'W'}  eul_statename={'phi', 'theta', 'psi'}  quat_statename={'qr', 'qi', 'qj','qk'}  pm_statename={'p', 'q', 'r'}  mass_statename=''
  Demux{1..6} (6 alike) : Demux  Outputs=3
  Gain : Gain  Gain=state.Mass
  Product : Product  Multiplication=Matrix(*)
  Sum2 : Sum  Inputs=++|  InputSameDT=on  SaturateOnIntegerOverflow=on  OutDataTypeStr=Inherit: Same as first input
  Terminator1 : Terminator
  Terminator2 : Terminator
  Bus Element Out3 : Outport  VectorParamsAs1DForOutWhenUnconnected=off  PortName=States  Element=Xe
  Bus Element Out4 : Outport  VectorParamsAs1DForOutWhenUnconnected=off  PortName=States  Element=Ze
  Bus Element Out : Outport  VectorParamsAs1DForOutWhenUnconnected=off  PortName=States  Element=theta
  Bus Element Out5 : Outport  VectorParamsAs1DForOutWhenUnconnected=off  PortName=States  Element=u
  Bus Element Out6 : Outport  VectorParamsAs1DForOutWhenUnconnected=off  PortName=States  Element=w
  Bus Element Out1 : Outport  VectorParamsAs1DForOutWhenUnconnected=off  PortName=States  Element=q
  Bus Element Out2 : Outport  VectorParamsAs1DForOutWhenUnconnected=off  PortName=States  Element=q_dot
  Bus Element Out7 : Outport  VectorParamsAs1DForOutWhenUnconnected=off  PortName=States  Element=Axe
  Bus Element Out8 : Outport  VectorParamsAs1DForOutWhenUnconnected=off  PortName=States  Element=Aze
  Bus Element Out15 : Outport  VectorParamsAs1DForOutWhenUnconnected=off  PortName=States  Element=Ye
  Bus Element Out9 : Outport  VectorParamsAs1DForOutWhenUnconnected=off  PortName=States  Element=phi
  Bus Element Out10 : Outport  VectorParamsAs1DForOutWhenUnconnected=off  PortName=States  Element=psi
  Bus Element Out16 : Outport  VectorParamsAs1DForOutWhenUnconnected=off  PortName=States  Element=v
  Bus Element Out11 : Outport  VectorParamsAs1DForOutWhenUnconnected=off  PortName=States  Element=p
  Bus Element Out12 : Outport  VectorParamsAs1DForOutWhenUnconnected=off  PortName=States  Element=r
  Bus Element Out13 : Outport  VectorParamsAs1DForOutWhenUnconnected=off  PortName=States  Element=p_dot
  Bus Element Out14 : Outport  VectorParamsAs1DForOutWhenUnconnected=off  PortName=States  Element=r_dot
  Bus Element Out17 : Outport  VectorParamsAs1DForOutWhenUnconnected=off  PortName=States  Element=Aye
  wires:
  6DOF (Euler Angles)/2 -> Demux1/1
  6DOF (Euler Angles)/4 -> Product/1
  6DOF (Euler Angles)/1 -> Terminator2/1
  Bus Element In/1 -> Gain/1
  Demux6/2 -> Bus Element Out17/1
  Demux6/3 -> Bus Element Out8/1
  Demux6/1 -> Bus Element Out7/1
  6DOF (Euler Angles)/9 -> Demux6/1
  6DOF (Euler Angles)/7 -> Demux5/1
  Demux5/3 -> Bus Element Out14/1
  Demux5/2 -> Bus Element Out2/1
  Demux5/1 -> Bus Element Out13/1
  6DOF (Euler Angles)/6 -> Demux4/1
  Demux4/3 -> Bus Element Out12/1
  Demux4/2 -> Bus Element Out1/1
  Demux4/1 -> Bus Element Out11/1
  Demux3/3 -> Bus Element Out6/1
  Demux3/2 -> Bus Element Out16/1
  Demux3/1 -> Bus Element Out5/1
  6DOF (Euler Angles)/5 -> Demux3/1
  Demux2/3 -> Bus Element Out10/1
  Demux2/2 -> Bus Element Out/1
  Demux2/1 -> Bus Element Out9/1
  Demux1/1 -> Bus Element Out3/1
  Demux1/3 -> Bus Element Out4/1
  Demux1/2 -> Bus Element Out15/1
  Gain/1 -> Product/2
  6DOF (Euler Angles)/3 -> Demux2/1
  Moments/1 -> 6DOF (Euler Angles)/2
  Forces/1 -> Sum2/2
  Sum2/1 -> 6DOF (Euler Angles)/1
  Product/1 -> Sum2/1
  6DOF (Euler Angles)/8 -> Terminator1/1

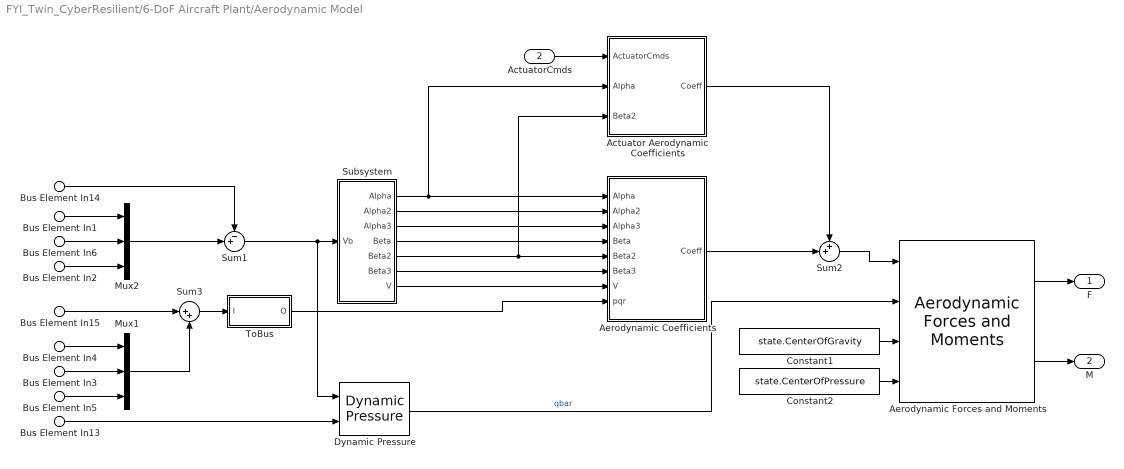
== system FYI_Twin_CyberResilient/6-DoF Aircraft Plant/Aerodynamic Model ==
  Bus Element In13 : Inport  PortName=Env  Element=AirDensity
  Bus Element In14 : Inport  PortName=Env  Element=WindVelocity
  Bus Element In15 : Inport  PortName=Env  Element=WindAngularRates
  ActuatorCmds : Inport  Port=2
  Bus Element In1 : Inport  Port=3  PortName=States  Element=u
  Bus Element In2 : Inport  Port=3  PortName=States  Element=w
  Bus Element In3 : Inport  Port=3  PortName=States  Element=q
  Bus Element In6 : Inport  Port=3  PortName=States  Element=v
  Bus Element In4 : Inport  Port=3  PortName=States  Element=p
  Bus Element In5 : Inport  Port=3  PortName=States  Element=r
  Actuator Aerodynamic Coefficients : Subsystem
  Aerodynamic Coefficients : Subsystem
  Aerodynamic Forces and Moments : aerolibadyn/Aerodynamic Forces and Moments   inputAxes=Body  outputForceAxes=Body  outputMomentAxes=Body  S=aircraft.ReferenceArea  b=aircraft.ReferenceSpan  cbar=aircraft.ReferenceLength
  Constant1 : Constant  Value=state.CenterOfGravity
  Constant2 : Constant  Value=state.CenterOfPressure
  Dynamic Pressure : aerolibasang/Dynamic Pressure
  Mux1 : Mux  Inputs=3
  Mux2 : Mux  Inputs=3
  Subsystem : Subsystem
  Sum1 : Sum  Inputs=-+|  InputSameDT=on  SaturateOnIntegerOverflow=on  OutDataTypeStr=Inherit: Same as first input
  Sum2 : Sum  Inputs=++|
  Sum3 : Sum  Inputs=|++  InputSameDT=on  SaturateOnIntegerOverflow=on  OutDataTypeStr=Inherit: Same as first input
  ToBus : Subsystem
  F : Outport  Unit=N  VectorParamsAs1DForOutWhenUnconnected=off
  M : Outport  Port=2  Unit=N*m  VectorParamsAs1DForOutWhenUnconnected=off
  wires:
  ActuatorCmds/1 -> Actuator Aerodynamic Coefficients/1(ActuatorCmds)
  Bus Element In14/1 -> Sum1/1
  Mux2/1 -> Sum1/2
  Mux1/1 -> Sum3/2
  Bus Element In15/1 -> Sum3/1
  Bus Element In5/1 -> Mux1/3
  Bus Element In3/1 -> Mux1/2
  Bus Element In4/1 -> Mux1/1
  Actuator Aerodynamic Coefficients/1(Coeff) -> Sum2/1
  Aerodynamic Coefficients/1(Coeff) -> Sum2/2
  ToBus/1(O) -> Aerodynamic Coefficients/8(pqr)
  Sum1/1 -> Dynamic Pressure/1, Subsystem/1(Vb)
  Dynamic Pressure/1 -> Aerodynamic Forces and Moments/2  "qbar"
  Sum3/1 -> ToBus/1(I)
  Bus Element In13/1 -> Dynamic Pressure/2
  Subsystem/7(V) -> Aerodynamic Coefficients/7(V)
  Subsystem/4(Beta) -> Aerodynamic Coefficients/4(Beta)
  Aerodynamic Forces and Moments/2 -> M/1
  Aerodynamic Forces and Moments/1 -> F/1
  Constant2/1 -> Aerodynamic Forces and Moments/4
  Constant1/1 -> Aerodynamic Forces and Moments/3
  Sum2/1 -> Aerodynamic Forces and Moments/1
  Bus Element In1/1 -> Mux2/1
  Bus Element In6/1 -> Mux2/2
  Bus Element In2/1 -> Mux2/3
  Subsystem/1(Alpha) -> Aerodynamic Coefficients/1(Alpha), Actuator Aerodynamic Coefficients/2(Alpha)
  Subsystem/5(Beta2) -> Aerodynamic Coefficients/5(Beta2), Actuator Aerodynamic Coefficients/3(Beta2)
  Subsystem/2(Alpha2) -> Aerodynamic Coefficients/2(Alpha2)
  Subsystem/3(Alpha3) -> Aerodynamic Coefficients/3(Alpha3)
  Subsystem/6(Beta3) -> Aerodynamic Coefficients/6(Beta3)

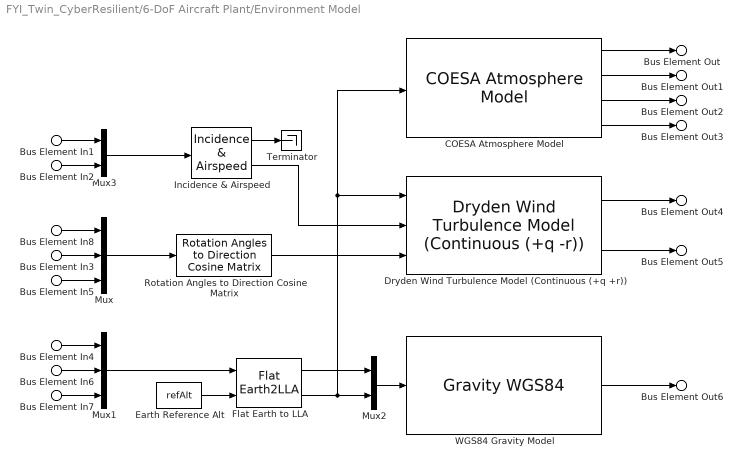
== system FYI_Twin_CyberResilient/6-DoF Aircraft Plant/Environment Model ==
  Bus Element In1 : Inport  PortName=States  Element=u
  Bus Element In2 : Inport  PortName=States  Element=w
  Bus Element In3 : Inport  PortName=States  Element=theta
  Bus Element In4 : Inport  PortName=States  Element=Xe
  Bus Element In7 : Inport  PortName=States  Element=Ze
  Bus Element In8 : Inport  PortName=States  Element=phi
  Bus Element In5 : Inport  PortName=States  Element=psi
  Bus Element In6 : Inport  PortName=States  Element=Ye
  COESA Atmosphere Model : aerolibatmos2/COESA Atmosphere Model  units=Metric (MKS)  spec=1976 COESA-extended U.S. Standard Atmosphere  model=Profile  profile_var=High temperature  profile_percent=1%  profile_alt=5 km (16404 ft)  envelope_var=High temperature  envelope_percent=1%  action=Warning
  Dryden Wind Turbulence Model (Continuous (+q +r)) : aerolibwind2/Dryden Wind Turbulence Model  (Continuous (+q -r))  units=Metric (MKS)  spec=MIL-F-8785C  model=Continuous Dryden (+q -r)  W20=W20  Wdeg=Wdeg  TurbProb=10^-2 - Light  L_high=L_high  Wingspan=Wingspan  ts=ts  Seed=Seed  T_on=on
  Earth Reference Alt : Constant  Value=refAlt
  Flat Earth to LLA : FlatEarth2LLA  R=6378137  LL0=[0 0]
  Incidence & Airspeed : aerolibasang/Incidence  & Airspeed
  Mux : Mux  Inputs=3
  Mux1 : Mux  Inputs=3
  Mux2 : Mux  Inputs=2
  Mux3 : Mux  Inputs=2
  Rotation Angles to Direction Cosine Matrix : sharedtransform/Rotation Angles to Direction Cosine Matrix  rotationOrder=ZYX  aMode=aMode
  Terminator : Terminator
  "WGS84 Gravity Model  " : GravityWGS84
  Bus Element Out : Outport  VectorParamsAs1DForOutWhenUnconnected=off  PortName=Env  Element=To
  Bus Element Out1 : Outport  VectorParamsAs1DForOutWhenUnconnected=off  PortName=Env  Element=a
  Bus Element Out2 : Outport  VectorParamsAs1DForOutWhenUnconnected=off  PortName=Env  Element=Po
  Bus Element Out3 : Outport  VectorParamsAs1DForOutWhenUnconnected=off  PortName=Env  Element=AirDensity
  Bus Element Out4 : Outport  VectorParamsAs1DForOutWhenUnconnected=off  PortName=Env  Element=WindVelocity
  Bus Element Out5 : Outport  VectorParamsAs1DForOutWhenUnconnected=off  PortName=Env  Element=WindAngularRates
  Bus Element Out6 : Outport  VectorParamsAs1DForOutWhenUnconnected=off  PortName=Env  Element=g
  wires:
  Dryden Wind Turbulence Model (Continuous (+q +r))/1 -> Bus Element Out4/1
  Dryden Wind Turbulence Model (Continuous (+q +r))/2 -> Bus Element Out5/1
  Mux2/1 -> "WGS84 Gravity Model  "/1
  Bus Element In4/1 -> Mux1/1
  Bus Element In7/1 -> Mux1/3
  Bus Element In6/1 -> Mux1/2
  Bus Element In5/1 -> Mux/3
  Bus Element In8/1 -> Mux/1
  Bus Element In2/1 -> Mux3/2
  Bus Element In1/1 -> Mux3/1
  "WGS84 Gravity Model  "/1 -> Bus Element Out6/1
  COESA Atmosphere Model/2 -> Bus Element Out1/1
  COESA Atmosphere Model/1 -> Bus Element Out/1
  COESA Atmosphere Model/4 -> Bus Element Out3/1
  COESA Atmosphere Model/3 -> Bus Element Out2/1
  Flat Earth to LLA/1 -> Mux2/1
  Earth Reference Alt/1 -> Flat Earth to LLA/2
  Incidence & Airspeed/2 -> Dryden Wind Turbulence Model (Continuous (+q +r))/2
  Flat Earth to LLA/2 -> Mux2/2, COESA Atmosphere Model/1, Dryden Wind Turbulence Model (Continuous (+q +r))/1
  Mux3/1 -> Incidence & Airspeed/1
  Incidence & Airspeed/1 -> Terminator/1
  Mux/1 -> Rotation Angles to Direction Cosine Matrix/1
  Bus Element In3/1 -> Mux/2
  Rotation Angles to Direction Cosine Matrix/1 -> Dryden Wind Turbulence Model (Continuous (+q +r))/3
  Mux1/1 -> Flat Earth to LLA/1

== system FYI_Twin_CyberResilient/6-DoF Aircraft Plant/Propulsion ==
  cmd : Inport
  Mux : Mux  Inputs=[1 2]
  ThrustX : Lookup_n-D  NumberOfTableDimensions=1  DataSpecification=Lookup table object  LookupTableObject=thrustX  BreakpointsForDimension1="getCoefficient(aircraft,\"CX\",\"Propeller\",Component=\"Propeller\").Breakpoints(1).Value"  IndexSearchMethod=Linear search  BeginIndexSearchUsingPreviousIndexResult=on  Table="getCoefficient(aircraft,\"CX\",\"Propeller\",Component=\"Propeller\").Table.Value"  ExtrapMethod=Clip
  ThrustYZ : Constant  Value=[0 0]'  SampleTime=-1
  Thrust_M1 : Constant  Value=[0 0 0]'  SampleTime=-1
  F : Outport  Unit=N  VectorParamsAs1DForOutWhenUnconnected=off
  M : Outport  Port=2  Unit=N*m  VectorParamsAs1DForOutWhenUnconnected=off
  wires:
  Thrust_M1/1 -> M/1
  ThrustX/1 -> Mux/1
  ThrustYZ/1 -> Mux/2
  Mux/1 -> F/1
  cmd/1 -> ThrustX/1

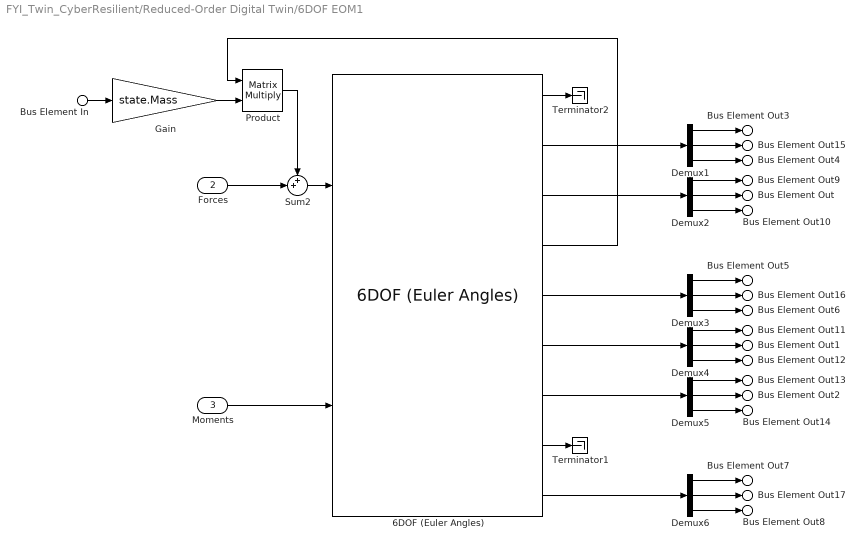
== system FYI_Twin_CyberResilient/Reduced-Order Digital Twin/6DOF EOM1 ==
  Bus Element In : Inport  PortName=Env  Element=g
  Forces : Inport  Port=2
  Moments : Inport  Port=3
  6DOF (Euler Angles) : aerolibobsolete/6DOF (Euler Angles)  units=Metric (MKS)  mtype=Fixed  rep=Euler Angles  xme_0=[Xe0, Ye0, Ze0]  Vm_0=[U0, V0, W0]  eul_0=[phi0, theta0, psi0]  pm_0=[p0, q0, r0]  mass_0=state.Mass  mass_e=0.5  mass_f=2.0  inertia=state.Inertia.Variables  inertia_e=eye(3)  inertia_f=2*eye(3)  k_quat=1.0  vre_flag=on  abi_flag=on  aMode=0  xme_statename={'Xe', 'Ye', 'Ze'}  Vm_statename={'U', 'V', 'W'}  eul_statename={'phi', 'theta', 'psi'}  quat_statename={'qr', 'qi', 'qj','qk'}  pm_statename={'p', 'q', 'r'}  mass_statename=''
  Demux{1..6} (6 alike) : Demux  Outputs=3
  Gain : Gain  Gain=state.Mass
  Product : Product  Multiplication=Matrix(*)
  Sum2 : Sum  Inputs=++|  InputSameDT=on  SaturateOnIntegerOverflow=on  OutDataTypeStr=Inherit: Same as first input
  Terminator1 : Terminator
  Terminator2 : Terminator
  Bus Element Out3 : Outport  VectorParamsAs1DForOutWhenUnconnected=off  PortName=States  Element=Xe
  Bus Element Out4 : Outport  VectorParamsAs1DForOutWhenUnconnected=off  PortName=States  Element=Ze
  Bus Element Out : Outport  VectorParamsAs1DForOutWhenUnconnected=off  PortName=States  Element=theta
  Bus Element Out5 : Outport  VectorParamsAs1DForOutWhenUnconnected=off  PortName=States  Element=u
  Bus Element Out6 : Outport  VectorParamsAs1DForOutWhenUnconnected=off  PortName=States  Element=w
  Bus Element Out1 : Outport  VectorParamsAs1DForOutWhenUnconnected=off  PortName=States  Element=q
  Bus Element Out2 : Outport  VectorParamsAs1DForOutWhenUnconnected=off  PortName=States  Element=q_dot
  Bus Element Out7 : Outport  VectorParamsAs1DForOutWhenUnconnected=off  PortName=States  Element=Axe
  Bus Element Out8 : Outport  VectorParamsAs1DForOutWhenUnconnected=off  PortName=States  Element=Aze
  Bus Element Out15 : Outport  VectorParamsAs1DForOutWhenUnconnected=off  PortName=States  Element=Ye
  Bus Element Out9 : Outport  VectorParamsAs1DForOutWhenUnconnected=off  PortName=States  Element=phi
  Bus Element Out10 : Outport  VectorParamsAs1DForOutWhenUnconnected=off  PortName=States  Element=psi
  Bus Element Out16 : Outport  VectorParamsAs1DForOutWhenUnconnected=off  PortName=States  Element=v
  Bus Element Out11 : Outport  VectorParamsAs1DForOutWhenUnconnected=off  PortName=States  Element=p
  Bus Element Out12 : Outport  VectorParamsAs1DForOutWhenUnconnected=off  PortName=States  Element=r
  Bus Element Out13 : Outport  VectorParamsAs1DForOutWhenUnconnected=off  PortName=States  Element=p_dot
  Bus Element Out14 : Outport  VectorParamsAs1DForOutWhenUnconnected=off  PortName=States  Element=r_dot
  Bus Element Out17 : Outport  VectorParamsAs1DForOutWhenUnconnected=off  PortName=States  Element=Aye
  wires:
  6DOF (Euler Angles)/2 -> Demux1/1
  6DOF (Euler Angles)/4 -> Product/1
  6DOF (Euler Angles)/1 -> Terminator2/1
  Bus Element In/1 -> Gain/1
  Demux6/2 -> Bus Element Out17/1
  Demux6/3 -> Bus Element Out8/1
  Demux6/1 -> Bus Element Out7/1
  6DOF (Euler Angles)/9 -> Demux6/1
  6DOF (Euler Angles)/7 -> Demux5/1
  Demux5/3 -> Bus Element Out14/1
  Demux5/2 -> Bus Element Out2/1
  Demux5/1 -> Bus Element Out13/1
  6DOF (Euler Angles)/6 -> Demux4/1
  Demux4/3 -> Bus Element Out12/1
  Demux4/2 -> Bus Element Out1/1
  Demux4/1 -> Bus Element Out11/1
  Demux3/3 -> Bus Element Out6/1
  Demux3/2 -> Bus Element Out16/1
  Demux3/1 -> Bus Element Out5/1
  6DOF (Euler Angles)/5 -> Demux3/1
  Demux2/3 -> Bus Element Out10/1
  Demux2/2 -> Bus Element Out/1
  Demux2/1 -> Bus Element Out9/1
  Demux1/1 -> Bus Element Out3/1
  Demux1/3 -> Bus Element Out4/1
  Demux1/2 -> Bus Element Out15/1
  Gain/1 -> Product/2
  6DOF (Euler Angles)/3 -> Demux2/1
  Moments/1 -> 6DOF (Euler Angles)/2
  Forces/1 -> Sum2/2
  Sum2/1 -> 6DOF (Euler Angles)/1
  Product/1 -> Sum2/1
  6DOF (Euler Angles)/8 -> Terminator1/1

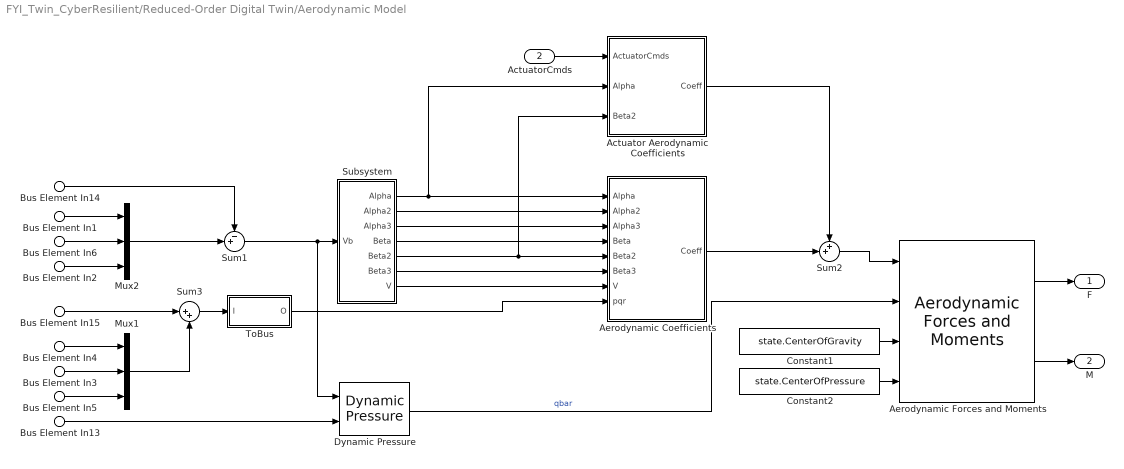
== system FYI_Twin_CyberResilient/Reduced-Order Digital Twin/Aerodynamic Model ==
  Bus Element In13 : Inport  PortName=Env  Element=AirDensity
  Bus Element In14 : Inport  PortName=Env  Element=WindVelocity
  Bus Element In15 : Inport  PortName=Env  Element=WindAngularRates
  ActuatorCmds : Inport  Port=2
  Bus Element In1 : Inport  Port=3  PortName=States  Element=u
  Bus Element In2 : Inport  Port=3  PortName=States  Element=w
  Bus Element In3 : Inport  Port=3  PortName=States  Element=q
  Bus Element In6 : Inport  Port=3  PortName=States  Element=v
  Bus Element In4 : Inport  Port=3  PortName=States  Element=p
  Bus Element In5 : Inport  Port=3  PortName=States  Element=r
  Actuator Aerodynamic Coefficients : Subsystem
  Aerodynamic Coefficients : Subsystem
  Aerodynamic Forces and Moments : aerolibadyn/Aerodynamic Forces and Moments   inputAxes=Body  outputForceAxes=Body  outputMomentAxes=Body  S=aircraft.ReferenceArea  b=aircraft.ReferenceSpan  cbar=aircraft.ReferenceLength
  Constant1 : Constant  Value=state.CenterOfGravity
  Constant2 : Constant  Value=state.CenterOfPressure
  Dynamic Pressure : aerolibasang/Dynamic Pressure
  Mux1 : Mux  Inputs=3
  Mux2 : Mux  Inputs=3
  Subsystem : Subsystem
  Sum1 : Sum  Inputs=-+|  InputSameDT=on  SaturateOnIntegerOverflow=on  OutDataTypeStr=Inherit: Same as first input
  Sum2 : Sum  Inputs=++|
  Sum3 : Sum  Inputs=|++  InputSameDT=on  SaturateOnIntegerOverflow=on  OutDataTypeStr=Inherit: Same as first input
  ToBus : Subsystem
  F : Outport  Unit=N  VectorParamsAs1DForOutWhenUnconnected=off
  M : Outport  Port=2  Unit=N*m  VectorParamsAs1DForOutWhenUnconnected=off
  wires:
  ActuatorCmds/1 -> Actuator Aerodynamic Coefficients/1(ActuatorCmds)
  Bus Element In14/1 -> Sum1/1
  Mux2/1 -> Sum1/2
  Mux1/1 -> Sum3/2
  Bus Element In15/1 -> Sum3/1
  Bus Element In5/1 -> Mux1/3
  Bus Element In3/1 -> Mux1/2
  Bus Element In4/1 -> Mux1/1
  Actuator Aerodynamic Coefficients/1(Coeff) -> Sum2/1
  Aerodynamic Coefficients/1(Coeff) -> Sum2/2
  ToBus/1(O) -> Aerodynamic Coefficients/8(pqr)
  Sum1/1 -> Dynamic Pressure/1, Subsystem/1(Vb)
  Dynamic Pressure/1 -> Aerodynamic Forces and Moments/2  "qbar"
  Sum3/1 -> ToBus/1(I)
  Bus Element In13/1 -> Dynamic Pressure/2
  Subsystem/7(V) -> Aerodynamic Coefficients/7(V)
  Subsystem/4(Beta) -> Aerodynamic Coefficients/4(Beta)
  Aerodynamic Forces and Moments/2 -> M/1
  Aerodynamic Forces and Moments/1 -> F/1
  Constant2/1 -> Aerodynamic Forces and Moments/4
  Constant1/1 -> Aerodynamic Forces and Moments/3
  Sum2/1 -> Aerodynamic Forces and Moments/1
  Bus Element In1/1 -> Mux2/1
  Bus Element In6/1 -> Mux2/2
  Bus Element In2/1 -> Mux2/3
  Subsystem/1(Alpha) -> Aerodynamic Coefficients/1(Alpha), Actuator Aerodynamic Coefficients/2(Alpha)
  Subsystem/5(Beta2) -> Aerodynamic Coefficients/5(Beta2), Actuator Aerodynamic Coefficients/3(Beta2)
  Subsystem/2(Alpha2) -> Aerodynamic Coefficients/2(Alpha2)
  Subsystem/3(Alpha3) -> Aerodynamic Coefficients/3(Alpha3)
  Subsystem/6(Beta3) -> Aerodynamic Coefficients/6(Beta3)
